simulink model "ForwardKinematic_YuMi"  (R2024a)
(part 21 of 23)

(3148506117433717*sin(q1R))/4503599627370496))/36893488147419103232 + sin(q2R)*((3148506117433717*cos(q1R))/4503599627370496 + (1211728953682539*sin(q1R))/2251799813685248)))/42535295865117307932921825928971026432))/1801439850948198400 - (94754841554645069948206780163139*sin(q5R)*(((7514214926474921*cos(q4R))/36893488147419103232 + (4503599440548691*sin(q4R))/4503599627370496)*((9007199067919185*sin(q3R)*((10914283902180054573281797610715*cos(q1R))/20282409603651670423947251286016 - (28359221366286827792295350160645*sin(q1R))/40564819207303340847894502572032))/9007199254740992 + cos(q3R)*(cos(q2R)*((3148506117433717*cos(q1R))/4503599627370496 + (1211728953682539*sin(q1R))/2251799813685248) - (7514214926474921*sin(q2R)*((1211728953682539*cos(q1R))/2251799813685248 - (3148506117433717*sin(q1R))/4503599627370496))/36893488147419103232) + (7514214926474921*sin(q3R)*((7514214926474921*cos(q2R)*((1211728953682539*cos(q1R))/2251799813685248 - (3148506117433717*sin(q1R))/4503599627370496))/36893488147419103232 + sin(q2R)*((3148506117433717*cos(q1R))/4503599627370496 + (1211728953682539*sin(q1R))/2251799813685248)))/36893488147419103232) + ((9007199067919185*cos(q4R))/9007199254740992 - (234819211581865*sin(q4R))/1152921504606846976)*((213097284493758984364555654519459856780913684045*sin(q1R))/1496577676626844588240573268701473812127674924007424 - (82012275009546312639155898108543355135168378515*cos(q1R))/748288838313422294120286634350736906063837462003712 + (67682029681889335677290557259385*cos(q2R)*((1211728953682539*cos(q1R))/2251799813685248 - (3148506117433717*sin(q1R))/4503599627370496))/332306998946228968225951765070086144 + (9007199067919185*sin(q2R)*((3148506117433717*cos(q1R))/4503599627370496 + (1211728953682539*sin(q1R))/2251799813685248))/9007199254740992) + (7514214926474921*sin(q4R)*((9007199067919185*cos(q3R)*((10914283902180054573281797610715*cos(q1R))/20282409603651670423947251286016 - (28359221366286827792295350160645*sin(q1R))/40564819207303340847894502572032))/9007199254740992 + (7514214926474921*cos(q3R)*((7514214926474921*cos(q2R)*((1211728953682539*cos(q1R))/2251799813685248 - (3148506117433717*sin(q1R))/4503599627370496))/36893488147419103232 + sin(q2R)*((3148506117433717*cos(q1R))/4503599627370496 + (1211728953682539*sin(q1R))/2251799813685248)))/36893488147419103232 - sin(q3R)*(cos(q2R)*((3148506117433717*cos(q1R))/4503599627370496 + (1211728953682539*sin(q1R))/2251799813685248) - (7514214926474921*sin(q2R)*((1211728953682539*cos(q1R))/2251799813685248 - (3148506117433717*sin(q1R))/4503599627370496))/36893488147419103232)))/36893488147419103232))/66461399789245793645190353014017228800 + (584133382113593486367040631332731*cos(q6R)*((965783844824089043900160825489639266458473927649494297144005158508529713680125*cos(q1R))/1042962419883256876169444192465601618458351817556959360325703910069443225478828393565899456512 - (2509452575434582988059840876067412966740105600591515474393999405526015293027875*sin(q1R))/2085924839766513752338888384931203236916703635113918720651407820138886450957656787131798913024 + (9007199067919185*((4503599440548691*cos(q4R))/4503599627370496 - (7514214926474921*sin(q4R))/36893488147419103232)*((9007199067919185*sin(q3R)*((10914283902180054573281797610715*cos(q1R))/20282409603651670423947251286016 - (28359221366286827792295350160645*sin(q1R))/40564819207303340847894502572032))/9007199254740992 + cos(q3R)*(cos(q2R)*((3148506117433717*cos(q1R))/4503599627370496 + (1211728953682539*sin(q1R))/2251799813685248) - (7514214926474921*sin(q2R)*((1211728953682539*cos(q1R))/2251799813685248 - (3148506117433717*sin(q1R))/4503599627370496))/36893488147419103232) + (7514214926474921*sin(q3R)*((7514214926474921*cos(q2R)*((1211728953682539*cos(q1R))/2251799813685248 - (3148506117433717*sin(q1R))/4503599627370496))/36893488147419103232 + sin(q2R)*((3148506117433717*cos(q1R))/4503599627370496 + (1211728953682539*sin(q1R))/2251799813685248)))/36893488147419103232))/9007199254740992 - (9007199067919185*((234819211581865*cos(q4R))/1152921504606846976 + (9007199067919185*sin(q4R))/9007199254740992)*((213097284493758984364555654519459856780913684045*sin(q1R))/1496577676626844588240573268701473812127674924007424 - (82012275009546312639155898108543355135168378515*cos(q1R))/748288838313422294120286634350736906063837462003712 + (67682029681889335677290557259385*cos(q2R)*((1211728953682539*cos(q1R))/2251799813685248 - (3148506117433717*sin(q1R))/4503599627370496))/332306998946228968225951765070086144 + (9007199067919185*sin(q2R)*((3148506117433717*cos(q1R))/4503599627370496 + (1211728953682539*sin(q1R))/2251799813685248))/9007199254740992))/9007199254740992 - (797029601289130257223357069404502671534492977261568326111352375*cos(q2R)*((1211728953682539*cos(q1R))/2251799813685248 - (3148506117433717*sin(q1R))/4503599627370496))/463168356949264781694283940034751631413079938662562256157830336031652518559744 - (106069577339469832923929692356850887620017617375*sin(q2R)*((3148506117433717*cos(q1R))/4503599627370496 + (1211728953682539*sin(q1R))/2251799813685248))/12554203470773361527671578846415332832204710888928069025792 + (67682029681889335677290557259385*cos(q4R)*((9007199067919185*cos(q3R)*((10914283902180054573281797610715*cos(q1R))/20282409603651670423947251286016 - (28359221366286827792295350160645*sin(q1R))/40564819207303340847894502572032))/9007199254740992 + (7514214926474921*cos(q3R)*((7514214926474921*cos(q2R)*((1211728953682539*cos(q1R))/2251799813685248 - (3148506117433717*sin(q1R))/4503599627370496))/36893488147419103232 + sin(q2R)*((3148506117433717*cos(q1R))/4503599627370496 + (1211728953682539*sin(q1R))/2251799813685248)))/36893488147419103232 - sin(q3R)*(cos(q2R)*((3148506117433717*cos(q1R))/4503599627370496 + (1211728953682539*sin(q1R))/2251799813685248) - (7514214926474921*sin(q2R)*((1211728953682539*cos(q1R))/2251799813685248 - (3148506117433717*sin(q1R))/4503599627370496))/36893488147419103232)))/332306998946228968225951765070086144 - (609625514665592237562888769449172969868262801225*cos(q3R)*((10914283902180054573281797610715*cos(q1R))/20282409603651670423947251286016 - (28359221366286827792295350160645*sin(q1R))/40564819207303340847894502572032))/2993155353253689176481146537402947624255349848014848 + (15893040848161638993908057577265778144967053025*sin(q3R)*((10914283902180054573281797610715*cos(q1R))/20282409603651670423947251286016 - (28359221366286827792295350160645*sin(q1R))/40564819207303340847894502572032))/383123885216472214589586756787577295904684780545900544 + (1764482024691522628700660907665*cos(q3R)*(cos(q2R)*((3148506117433717*cos(q1R))/4503599627370496 + (1211728953682539*sin(q1R))/2251799813685248) - (7514214926474921*sin(q2R)*((1211728953682539*cos(q1R))/2251799813685248 - (3148506117433717*sin(q1R))/4503599627370496))/36893488147419103232))/42535295865117307932921825928971026432 - (508577317689771495245073589786522929324694383585*cos(q3R)*((7514214926474921*cos(q2R)*((1211728953682539*cos(q1R))/2251799813685248 - (3148506117433717*sin(q1R))/4503599627370496))/36893488147419103232 + sin(q2R)*((3148506117433717*cos(q1R))/4503599627370496 + (1211728953682539*sin(q1R))/2251799813685248)))/12259964326927110866866776217202473468949912977468817408 + (67682029681889335677290557259385*sin(q3R)*(cos(q2R)*((3148506117433717*cos(q1R))/4503599627370496 + (1211728953682539*sin(q1R))/2251799813685248) - (7514214926474921*sin(q2R)*((1211728953682539*cos(q1R))/2251799813685248 - (3148506117433717*sin(q1R))/4503599627370496))/36893488147419103232))/332306998946228968225951765070086144 + (13258697167433729449897784796786197386719169465*sin(q3R)*((7514214926474921*cos(q2R)*((1211728953682539*cos(q1R))/2251799813685248 - (3148506117433717*sin(q1R))/4503599627370496))/36893488147419103232 + sin(q2R)*((3148506117433717*cos(q1R))/4503599627370496 + (1211728953682539*sin(q1R))/2251799813685248)))/1569275433846670190958947355801916604025588861116008628224))/16225927682921336339157801028812800 + (48638874966763599*sin(q6R)*((965783844824089043900160825489639266458473927649494297144005158508529713680125*cos(q1R))/1042962419883256876169444192465601618458351817556959360325703910069443225478828393565899456512 - (2509452575434582988059840876067412966740105600591515474393999405526015293027875*sin(q1R))/2085924839766513752338888384931203236916703635113918720651407820138886450957656787131798913024 + (9007199067919185*((4503599440548691*cos(q4R))/4503599627370496 - (7514214926474921*sin(q4R))/36893488147419103232)*((9007199067919185*sin(q3R)*((10914283902180054573281797610715*cos(q1R))/20282409603651670423947251286016 - (28359221366286827792295350160645*sin(q1R))/40564819207303340847894502572032))/9007199254740992 + cos(q3R)*(cos(q2R)*((3148506117433717*cos(q1R))/4503599627370496 + (1211728953682539*sin(q1R))/2251799813685248) - (7514214926474921*sin(q2R)*((1211728953682539*cos(q1R))/2251799813685248 - (3148506117433717*sin(q1R))/4503599627370496))/36893488147419103232) + (7514214926474921*sin(q3R)*((7514214926474921*cos(q2R)*((1211728953682539*cos(q1R))/2251799813685248 - (3148506117433717*sin(q1R))/4503599627370496))/36893488147419103232 + sin(q2R)*((3148506117433717*cos(q1R))/4503599627370496 + (1211728953682539*sin(q1R))/2251799813685248)))/36893488147419103232))/9007199254740992 - (9007199067919185*((234819211581865*cos(q4R))/1152921504606846976 + (9007199067919185*sin(q4R))/9007199254740992)*((213097284493758984364555654519459856780913684045*sin(q1R))/1496577676626844588240573268701473812127674924007424 - (82012275009546312639155898108543355135168378515*cos(q1R))/748288838313422294120286634350736906063837462003712 + (67682029681889335677290557259385*cos(q2R)*((1211728953682539*cos(q1R))/2251799813685248 - (3148506117433717*sin(q1R))/4503599627370496))/332306998946228968225951765070086144 + (9007199067919185*sin(q2R)*((3148506117433717*cos(q1R))/4503599627370496 + (1211728953682539*sin(q1R))/2251799813685248))/9007199254740992))/9007199254740992 - (797029601289130257223357069404502671534492977261568326111352375*cos(q2R)*((1211728953682539*cos(q1R))/2251799813685248 - (3148506117433717*sin(q1R))/4503599627370496))/463168356949264781694283940034751631413079938662562256157830336031652518559744 - (106069577339469832923929692356850887620017617375*sin(q2R)*((3148506117433717*cos(q1R))/4503599627370496 + (1211728953682539*sin(q1R))/2251799813685248))/12554203470773361527671578846415332832204710888928069025792 + (67682029681889335677290557259385*cos(q4R)*((9007199067919185*cos(q3R)*((10914283902180054573281797610715*cos(q1R))/20282409603651670423947251286016 - (28359221366286827792295350160645*sin(q1R))/40564819207303340847894502572032))/9007199254740992 + (7514214926474921*cos(q3R)*((7514214926474921*cos(q2R)*((1211728953682539*cos(q1R))/2251799813685248 - (3148506117433717*sin(q1R))/4503599627370496))/36893488147419103232 + sin(q2R)*((3148506117433717*cos(q1R))/4503599627370496 + (1211728953682539*sin(q1R))/2251799813685248)))/36893488147419103232 - sin(q3R)*(cos(q2R)*((3148506117433717*cos(q1R))/4503599627370496 + (1211728953682539*sin(q1R))/2251799813685248) - (7514214926474921*sin(q2R)*((1211728953682539*cos(q1R))/2251799813685248 - (3148506117433717*sin(q1R))/4503599627370496))/36893488147419103232)))/332306998946228968225951765070086144 - (609625514665592237562888769449172969868262801225*cos(q3R)*((10914283902180054573281797610715*cos(q1R))/20282409603651670423947251286016 - (28359221366286827792295350160645*sin(q1R))/40564819207303340847894502572032))/2993155353253689176481146537402947624255349848014848 + (15893040848161638993908057577265778144967053025*sin(q3R)*((10914283902180054573281797610715*cos(q1R))/20282409603651670423947251286016 - (28359221366286827792295350160645*sin(q1R))/40564819207303340847894502572032))/383123885216472214589586756787577295904684780545900544 + (1764482024691522628700660907665*cos(q3R)*(cos(q2R)*((3148506117433717*cos(q1R))/4503599627370496 + (1211728953682539*sin(q1R))/2251799813685248) - (7514214926474921*sin(q2R)*((1211728953682539*cos(q1R))/2251799813685248 - (3148506117433717*sin(q1R))/4503599627370496))/36893488147419103232))/42535295865117307932921825928971026432 - (508577317689771495245073589786522929324694383585*cos(q3R)*((7514214926474921*cos(q2R)*((1211728953682539*cos(q1R))/2251799813685248 - (3148506117433717*sin(q1R))/4503599627370496))/36893488147419103232 + sin(q2R)*((3148506117433717*cos(q1R))/4503599627370496 + (1211728953682539*sin(q1R))/2251799813685248)))/12259964326927110866866776217202473468949912977468817408 + (67682029681889335677290557259385*sin(q3R)*(cos(q2R)*((3148506117433717*cos(q1R))/4503599627370496 + (1211728953682539*sin(q1R))/2251799813685248) - (7514214926474921*sin(q2R)*((1211728953682539*cos(q1R))/2251799813685248 - (3148506117433717*sin(q1R))/4503599627370496))/36893488147419103232))/332306998946228968225951765070086144 + (13258697167433729449897784796786197386719169465*sin(q3R)*((7514214926474921*cos(q2R)*((1211728953682539*cos(q1R))/2251799813685248 - (3148506117433717*sin(q1R))/4503599627370496))/36893488147419103232 + sin(q2R)*((3148506117433717*cos(q1R))/4503599627370496 + (1211728953682539*sin(q1R))/2251799813685248)))/1569275433846670190958947355801916604025588861116008628224))/1801439850948198400 + (610321541873521657855151997354401418608858870661075444886782706002880706727*cos(q4R)*((9007199067919185*cos(q3R)*((10914283902180054573281797610715*cos(q1R))/20282409603651670423947251286016 - (28359221366286827792295350160645*sin(q1R))/40564819207303340847894502572032))/9007199254740992 + (7514214926474921*cos(q3R)*((7514214926474921*cos(q2R)*((1211728953682539*cos(q1R))/2251799813685248 - (3148506117433717*sin(q1R))/4503599627370496))/36893488147419103232 + sin(q2R)*((3148506117433717*cos(q1R))/4503599627370496 + (1211728953682539*sin(q1R))/2251799813685248)))/36893488147419103232 - sin(q3R)*(cos(q2R)*((3148506117433717*cos(q1R))/4503599627370496 + (1211728953682539*sin(q1R))/2251799813685248) - (7514214926474921*sin(q2R)*((1211728953682539*cos(q1R))/2251799813685248 - (3148506117433717*sin(q1R))/4503599627370496))/36893488147419103232)))/11307821214581659709333104004754678501295896940003961331978279688272766566400000 + (608651409044468601*sin(q4R)*((9007199067919185*cos(q3R)*((10914283902180054573281797610715*cos(q1R))/20282409603651670423947251286016 - (28359221366286827792295350160645*sin(q1R))/40564819207303340847894502572032))/9007199254740992 + (7514214926474921*cos(q3R)*((7514214926474921*cos(q2R)*((1211728953682539*cos(q1R))/2251799813685248 - (3148506117433717*sin(q1R))/4503599627370496))/36893488147419103232 + sin(q2R)*((3148506117433717*cos(q1R))/4503599627370496 + (1211728953682539*sin(q1R))/2251799813685248)))/36893488147419103232 - sin(q3R)*(cos(q2R)*((3148506117433717*cos(q1R))/4503599627370496 + (1211728953682539*sin(q1R))/2251799813685248) - (7514214926474921*sin(q2R)*((1211728953682539*cos(q1R))/2251799813685248 - (3148506117433717*sin(q1R))/4503599627370496))/36893488147419103232)))/73786976294838206464000 - (83301539375654672537075965313343183841442266989297270401707771044036658496661398777306991*cos(q3R)*((10914283902180054573281797610715*cos(q1R))/20282409603651670423947251286016 - (28359221366286827792295350160645*sin(q1R))/40564819207303340847894502572032))/4074071952668972172536891376818756322102936787331872501272280898708762599526673412366794752000 + (109198173955282063961996941994332957526645881091499469714283881779231664456243735535448036415347*sin(q3R)*((10914283902180054573281797610715*cos(q1R))/20282409603651670423947251286016 - (28359221366286827792295350160645*sin(q1R))/40564819207303340847894502572032))/2607406049708142190423610481164004046145879543892398400814259775173608063697070983914748641280000 + (60617164743372705924380750591060836759586313939367162716784907429017787816377231*cos(q3R)*(cos(q2R)*((3148506117433717*cos(q1R))/4503599627370496 + (1211728953682539*sin(q1R))/2251799813685248) - (7514214926474921*sin(q2R)*((1211728953682539*cos(q1R))/2251799813685248 - (3148506117433717*sin(q1R))/4503599627370496))/36893488147419103232))/1447401115466452442794637312608598848165874808320507050493219800098914120499200000 - (347469655025336708709976918716104493695816557877713443586884917071777956519687017125887603*cos(q3R)*((7514214926474921*cos(q2R)*((1211728953682539*cos(q1R))/2251799813685248 - (3148506117433717*sin(q1R))/4503599627370496))/36893488147419103232 + sin(q2R)*((3148506117433717*cos(q1R))/4503599627370496 + (1211728953682539*sin(q1R))/2251799813685248)))/83436993590660550093555535397248129476668145404556748826056312805555458038306271485271956520960000 + (46241644459901303158631016767207157814229090534989303509431886332469146043*sin(q3R)*(cos(q2R)*((3148506117433717*cos(q1R))/4503599627370496 + (1211728953682539*sin(q1R))/2251799813685248) - (7514214926474921*sin(q2R)*((1211728953682539*cos(q1R))/2251799813685248 - (3148506117433717*sin(q1R))/4503599627370496))/36893488147419103232))/2261564242916331941866620800950935700259179388000792266395655937654553313280000 + (455490404115240510935077772268745492204390157443214084883134054419271951750419293234291596923751*sin(q3R)*((7514214926474921*cos(q2R)*((1211728953682539*cos(q1R))/2251799813685248 - (3148506117433717*sin(q1R))/4503599627370496))/36893488147419103232 + sin(q2R)*((3148506117433717*cos(q1R))/4503599627370496 + (1211728953682539*sin(q1R))/2251799813685248)))/53399675898022752059875542654238802865067613058916319248676040195555493144516013750574052173414400000, (81222263116692158804177042061221826384594597321566869716687*((234819211581865*cos(q4R))/1152921504606846976 + (9007199067919185*sin(q4R))/9007199254740992)*((43007175577195104036898489188735438973874147925*sin(q2R))/91343852333181432387730302044767688728495783936 + (9007199067919185*cos(q2R)*((1211728953682539*cos(q1R))/2251799813685248 - (3148506117433717*sin(q1R))/4503599627370496))/9007199254740992 + (67682029681889335677290557259385*sin(q2R)*((3148506117433717*cos(q1R))/4503599627370496 + (1211728953682539*sin(q1R))/2251799813685248))/332306998946228968225951765070086144))/306499108173177771671669405430061836723747824436720435200000 - (102624569379093796004717602421110099184671668506065630314089972323079075980539460999909738524689495122204956357382384585416279829311*sin(q2R))/866459279412754643618254432544713657323886586054942679740774868942069158689258007199992001907543618155434753425438616196554424320000 - (610321541873521657855151997354401418608858870661075444886782706002880706727*cos(q4R)*((7514214926474921*cos(q3R)*((4774755754024928798560446539205*sin(q2R))/10141204801825835211973625643008 + cos(q2R)*((1211728953682539*cos(q1R))/2251799813685248 - (3148506117433717*sin(q1R))/4503599627370496) + (7514214926474921*sin(q2R)*((3148506117433717*cos(q1R))/4503599627370496 + (1211728953682539*sin(q1R))/2251799813685248))/36893488147419103232))/36893488147419103232 - sin(q3R)*((4774755754024928798560446539205*cos(q2R))/10141204801825835211973625643008 + (7514214926474921*cos(q2R)*((3148506117433717*cos(q1R))/4503599627370496 + (1211728953682539*sin(q1R))/2251799813685248))/36893488147419103232 - sin(q2R)*((1211728953682539*cos(q1R))/2251799813685248 - (3148506117433717*sin(q1R))/4503599627370496))))/11307821214581659709333104004754678501295896940003961331978279688272766566400000 - (608651409044468601*sin(q4R)*((7514214926474921*cos(q3R)*((4774755754024928798560446539205*sin(q2R))/10141204801825835211973625643008 + cos(q2R)*((1211728953682539*cos(q1R))/2251799813685248 - (3148506117433717*sin(q1R))/4503599627370496) + (7514214926474921*sin(q2R)*((3148506117433717*cos(q1R))/4503599627370496 + (1211728953682539*sin(q1R))/2251799813685248))/36893488147419103232))/36893488147419103232 - sin(q3R)*((4774755754024928798560446539205*cos(q2R))/10141204801825835211973625643008 + (7514214926474921*cos(q2R)*((3148506117433717*cos(q1R))/4503599627370496 + (1211728953682539*sin(q1R))/2251799813685248))/36893488147419103232 - sin(q2R)*((1211728953682539*cos(q1R))/2251799813685248 - (3148506117433717*sin(q1R))/4503599627370496))))/73786976294838206464000 - (81*((9007199067919185*cos(q4R))/9007199254740992 - (234819211581865*sin(q4R))/1152921504606846976)*((43007175577195104036898489188735438973874147925*sin(q2R))/91343852333181432387730302044767688728495783936 + (9007199067919185*cos(q2R)*((1211728953682539*cos(q1R))/2251799813685248 - (3148506117433717*sin(q1R))/4503599627370496))/9007199254740992 + (67682029681889335677290557259385*sin(q2R)*((3148506117433717*cos(q1R))/4503599627370496 + (1211728953682539*sin(q1R))/2251799813685248))/332306998946228968225951765070086144))/2000 - (2864853452414957279136267923523*cos(q2R))/202824096036516704239472512860160 + (170695144106365826517608855445768431563113584343*cos(q5R)*((67399765602155231606998903473897443684277400996768941497011875*sin(q2R))/3450873173395281893717377931138512726225554486085193277581262111899648 + (14115856197532180673579726082375*cos(q2R)*((1211728953682539*cos(q1R))/2251799813685248 - (3148506117433717*sin(q1R))/4503599627370496))/340282366920938463463374607431768211456 - (234819211581865*cos(q3R)*((4774755754024928798560446539205*cos(q2R))/10141204801825835211973625643008 + (7514214926474921*cos(q2R)*((3148506117433717*cos(q1R))/4503599627370496 + (1211728953682539*sin(q1R))/2251799813685248))/36893488147419103232 - sin(q2R)*((1211728953682539*cos(q1R))/2251799813685248 - (3148506117433717*sin(q1R))/4503599627370496)))/1152921504606846976 + (106069577339469832923929692356850887620017617375*sin(q2R)*((3148506117433717*cos(q1R))/4503599627370496 + (1211728953682539*sin(q1R))/2251799813685248))/12554203470773361527671578846415332832204710888928069025792 + (67682029681889335677290557259385*cos(q3R)*((4774755754024928798560446539205*sin(q2R))/10141204801825835211973625643008 + cos(q2R)*((1211728953682539*cos(q1R))/2251799813685248 - (3148506117433717*sin(q1R))/4503599627370496) + (7514214926474921*sin(q2R)*((3148506117433717*cos(q1R))/4503599627370496 + (1211728953682539*sin(q1R))/2251799813685248))/36893488147419103232))/332306998946228968225951765070086144 - (9007199067919185*sin(q3R)*((4774755754024928798560446539205*cos(q2R))/10141204801825835211973625643008 + (7514214926474921*cos(q2R)*((3148506117433717*cos(q1R))/4503599627370496 + (1211728953682539*sin(q1R))/2251799813685248))/36893488147419103232 - sin(q2R)*((1211728953682539*cos(q1R))/2251799813685248 - (3148506117433717*sin(q1R))/4503599627370496)))/9007199254740992 - (1764482024691522628700660907665*sin(q3R)*((4774755754024928798560446539205*sin(q2R))/10141204801825835211973625643008 + cos(q2R)*((1211728953682539*cos(q1R))/2251799813685248 - (3148506117433717*sin(q1R))/4503599627370496) + (7514214926474921*sin(q2R)*((3148506117433717*cos(q1R))/4503599627370496 + (1211728953682539*sin(q1R))/2251799813685248))/36893488147419103232))/42535295865117307932921825928971026432))/119726214130147567059245861496117904970213993920593920 - (48638874966763599*sin(q5R)*((67399765602155231606998903473897443684277400996768941497011875*sin(q2R))/3450873173395281893717377931138512726225554486085193277581262111899648 + (14115856197532180673579726082375*cos(q2R)*((1211728953682539*cos(q1R))/2251799813685248 - (3148506117433717*sin(q1R))/4503599627370496))/340282366920938463463374607431768211456 - (234819211581865*cos(q3R)*((4774755754024928798560446539205*cos(q2R))/10141204801825835211973625643008 + (7514214926474921*cos(q2R)*((3148506117433717*cos(q1R))/4503599627370496 + (1211728953682539*sin(q1R))/2251799813685248))/36893488147419103232 - sin(q2R)*((1211728953682539*cos(q1R))/2251799813685248 - (3148506117433717*sin(q1R))/4503599627370496)))/1152921504606846976 + (106069577339469832923929692356850887620017617375*sin(q2R)*((3148506117433717*cos(q1R))/4503599627370496 + (1211728953682539*sin(q1R))/2251799813685248))/12554203470773361527671578846415332832204710888928069025792 + (67682029681889335677290557259385*cos(q3R)*((4774755754024928798560446539205*sin(q2R))/10141204801825835211973625643008 + cos(q2R)*((1211728953682539*cos(q1R))/2251799813685248 - (3148506117433717*sin(q1R))/4503599627370496) + (7514214926474921*sin(q2R)*((3148506117433717*cos(q1R))/4503599627370496 + (1211728953682539*sin(q1R))/2251799813685248))/36893488147419103232))/332306998946228968225951765070086144 - (9007199067919185*sin(q3R)*((4774755754024928798560446539205*cos(q2R))/10141204801825835211973625643008 + (7514214926474921*cos(q2R)*((3148506117433717*cos(q1R))/4503599627370496 + (1211728953682539*sin(q1R))/2251799813685248))/36893488147419103232 - sin(q2R)*((1211728953682539*cos(q1R))/2251799813685248 - (3148506117433717*sin(q1R))/4503599627370496)))/9007199254740992 - (1764482024691522628700660907665*sin(q3R)*((4774755754024928798560446539205*sin(q2R))/10141204801825835211973625643008 + cos(q2R)*((1211728953682539*cos(q1R))/2251799813685248 - (3148506117433717*sin(q1R))/4503599627370496) + (7514214926474921*sin(q2R)*((3148506117433717*cos(q1R))/4503599627370496 + (1211728953682539*sin(q1R))/2251799813685248))/36893488147419103232))/42535295865117307932921825928971026432))/1801439850948198400 - (107465779053290185796889472867275736954369330186921663479979246519176992895505610212310958309481948671*cos(q2R)*((1211728953682539*cos(q1R))/2251799813685248 - (3148506117433717*sin(q1R))/4503599627370496))/427197407184182016479004341233910422920540904471330553989408321564443945156128110004592417387315200000 - (22542644779424763*cos(q2R)*((3148506117433717*cos(q1R))/4503599627370496 + (1211728953682539*sin(q1R))/2251799813685248))/3689348814741910323200 - (60617164743372705924380750591060836759586313939367162716784907429017787816377231*cos(q3R)*((4774755754024928798560446539205*cos(q2R))/10141204801825835211973625643008 + (7514214926474921*cos(q2R)*((3148506117433717*cos(q1R))/4503599627370496 + (1211728953682539*sin(q1R))/2251799813685248))/36893488147419103232 - sin(q2R)*((1211728953682539*cos(q1R))/2251799813685248 - (3148506117433717*sin(q1R))/4503599627370496)))/1447401115466452442794637312608598848165874808320507050493219800098914120499200000 + (3*sin(q2R)*((1211728953682539*cos(q1R))/2251799813685248 - (3148506117433717*sin(q1R))/4503599627370496))/100 - (807520961047489018778067709720399904923771262077295170375712179706208528987338271217011451790113918662491539890779991*sin(q2R)*((3148506117433717*cos(q1R))/4503599627370496 + (1211728953682539*sin(q1R))/2251799813685248))/15760802478557791684911616040057445522031895708186178667179317361698288708598884244565706501953966256322651196122726400000 + (347469655025336708709976918716104493695816557877713443586884917071777956519687017125887603*cos(q3R)*((4774755754024928798560446539205*sin(q2R))/10141204801825835211973625643008 + cos(q2R)*((1211728953682539*cos(q1R))/2251799813685248 - (3148506117433717*sin(q1R))/4503599627370496) + (7514214926474921*sin(q2R)*((3148506117433717*cos(q1R))/4503599627370496 + (1211728953682539*sin(q1R))/2251799813685248))/36893488147419103232))/83436993590660550093555535397248129476668145404556748826056312805555458038306271485271956520960000 - (46241644459901303158631016767207157814229090534989303509431886332469146043*sin(q3R)*((4774755754024928798560446539205*cos(q2R))/10141204801825835211973625643008 + (7514214926474921*cos(q2R)*((3148506117433717*cos(q1R))/4503599627370496 + (1211728953682539*sin(q1R))/2251799813685248))/36893488147419103232 - sin(q2R)*((1211728953682539*cos(q1R))/2251799813685248 - (3148506117433717*sin(q1R))/4503599627370496)))/2261564242916331941866620800950935700259179388000792266395655937654553313280000 - (81222263116692158804177042061221826384594597321566869716687*((4503599440548691*cos(q4R))/4503599627370496 - (7514214926474921*sin(q4R))/36893488147419103232)*(cos(q3R)*((4774755754024928798560446539205*cos(q2R))/10141204801825835211973625643008 + (7514214926474921*cos(q2R)*((3148506117433717*cos(q1R))/4503599627370496 + (1211728953682539*sin(q1R))/2251799813685248))/36893488147419103232 - sin(q2R)*((1211728953682539*cos(q1R))/2251799813685248 - (3148506117433717*sin(q1R))/4503599627370496)) + (7514214926474921*sin(q3R)*((4774755754024928798560446539205*sin(q2R))/10141204801825835211973625643008 + cos(q2R)*((1211728953682539*cos(q1R))/2251799813685248 - (3148506117433717*sin(q1R))/4503599627370496) + (7514214926474921*sin(q2R)*((3148506117433717*cos(q1R))/4503599627370496 + (1211728953682539*sin(q1R))/2251799813685248))/36893488147419103232))/36893488147419103232))/306499108173177771671669405430061836723747824436720435200000 - (81*((7514214926474921*cos(q4R))/36893488147419103232 + (4503599440548691*sin(q4R))/4503599627370496)*(cos(q3R)*((4774755754024928798560446539205*cos(q2R))/10141204801825835211973625643008 + (7514214926474921*cos(q2R)*((3148506117433717*cos(q1R))/4503599627370496 + (1211728953682539*sin(q1R))/2251799813685248))/36893488147419103232 - sin(q2R)*((1211728953682539*cos(q1R))/2251799813685248 - (3148506117433717*sin(q1R))/4503599627370496)) + (7514214926474921*sin(q3R)*((4774755754024928798560446539205*sin(q2R))/10141204801825835211973625643008 + cos(q2R)*((1211728953682539*cos(q1R))/2251799813685248 - (3148506117433717*sin(q1R))/4503599627370496) + (7514214926474921*sin(q2R)*((3148506117433717*cos(q1R))/4503599627370496 + (1211728953682539*sin(q1R))/2251799813685248))/36893488147419103232))/36893488147419103232))/2000 - (455490404115240510935077772268745492204390157443214084883134054419271951750419293234291596923751*sin(q3R)*((4774755754024928798560446539205*sin(q2R))/10141204801825835211973625643008 + cos(q2R)*((1211728953682539*cos(q1R))/2251799813685248 - (3148506117433717*sin(q1R))/4503599627370496) + (7514214926474921*sin(q2R)*((3148506117433717*cos(q1R))/4503599627370496 + (1211728953682539*sin(q1R))/2251799813685248))/36893488147419103232))/53399675898022752059875542654238802865067613058916319248676040195555493144516013750574052173414400000 + (712008244765680093343103025701132101054572137019*cos(q5R)*((7514214926474921*cos(q4R)*((7514214926474921*cos(q3R)*((4774755754024928798560446539205*sin(q2R))/10141204801825835211973625643008 + cos(q2R)*((1211728953682539*cos(q1R))/2251799813685248 - (3148506117433717*sin(q1R))/4503599627370496) + (7514214926474921*sin(q2R)*((3148506117433717*cos(q1R))/4503599627370496 + (1211728953682539*sin(q1R))/2251799813685248))/36893488147419103232))/36893488147419103232 - sin(q3R)*((4774755754024928798560446539205*cos(q2R))/10141204801825835211973625643008 + (7514214926474921*cos(q2R)*((3148506117433717*cos(q1R))/4503599627370496 + (1211728953682539*sin(q1R))/2251799813685248))/36893488147419103232 - sin(q2R)*((1211728953682539*cos(q1R))/2251799813685248 - (3148506117433717*sin(q1R))/4503599627370496))))/36893488147419103232 - ((234819211581865*cos(q4R))/1152921504606846976 + (9007199067919185*sin(q4R))/9007199254740992)*((43007175577195104036898489188735438973874147925*sin(q2R))/91343852333181432387730302044767688728495783936 + (9007199067919185*cos(q2R)*((1211728953682539*cos(q1R))/2251799813685248 - (3148506117433717*sin(q1R))/4503599627370496))/9007199254740992 + (67682029681889335677290557259385*sin(q2R)*((3148506117433717*cos(q1R))/4503599627370496 + (1211728953682539*sin(q1R))/2251799813685248))/332306998946228968225951765070086144) + ((4503599440548691*cos(q4R))/4503599627370496 - (7514214926474921*sin(q4R))/36893488147419103232)*(cos(q3R)*((4774755754024928798560446539205*cos(q2R))/10141204801825835211973625643008 + (7514214926474921*cos(q2R)*((3148506117433717*cos(q1R))/4503599627370496 + (1211728953682539*sin(q1R))/2251799813685248))/36893488147419103232 - sin(q2R)*((1211728953682539*cos(q1R))/2251799813685248 - (3148506117433717*sin(q1R))/4503599627370496)) + (7514214926474921*sin(q3R)*((4774755754024928798560446539205*sin(q2R))/10141204801825835211973625643008 + cos(q2R)*((1211728953682539*cos(q1R))/2251799813685248 - (3148506117433717*sin(q1R))/4503599627370496) + (7514214926474921*sin(q2R)*((3148506117433717*cos(q1R))/4503599627370496 + (1211728953682539*sin(q1R))/2251799813685248))/36893488147419103232))/36893488147419103232)))/2451992865385422173373355243440494693789982595493763481600 - (2436553109258773196144549622003023*cos(q6R)*((9007199067919185*cos(q5R)*((67399765602155231606998903473897443684277400996768941497011875*sin(q2R))/3450873173395281893717377931138512726225554486085193277581262111899648 + (14115856197532180673579726082375*cos(q2R)*((1211728953682539*cos(q1R))/2251799813685248 - (3148506117433717*sin(q1R))/4503599627370496))/340282366920938463463374607431768211456 - (234819211581865*cos(q3R)*((4774755754024928798560446539205*cos(q2R))/10141204801825835211973625643008 + (7514214926474921*cos(q2R)*((3148506117433717*cos(q1R))/4503599627370496 + (1211728953682539*sin(q1R))/2251799813685248))/36893488147419103232 - sin(q2R)*((1211728953682539*cos(q1R))/2251799813685248 - (3148506117433717*sin(q1R))/4503599627370496)))/1152921504606846976 + (106069577339469832923929692356850887620017617375*sin(q2R)*((3148506117433717*cos(q1R))/4503599627370496 + (1211728953682539*sin(q1R))/2251799813685248))/12554203470773361527671578846415332832204710888928069025792 + (67682029681889335677290557259385*cos(q3R)*((4774755754024928798560446539205*sin(q2R))/10141204801825835211973625643008 + cos(q2R)*((1211728953682539*cos(q1R))/2251799813685248 - (3148506117433717*sin(q1R))/4503599627370496) + (7514214926474921*sin(q2R)*((3148506117433717*cos(q1R))/4503599627370496 + (1211728953682539*sin(q1R))/2251799813685248))/36893488147419103232))/332306998946228968225951765070086144 - (9007199067919185*sin(q3R)*((4774755754024928798560446539205*cos(q2R))/10141204801825835211973625643008 + (7514214926474921*cos(q2R)*((3148506117433717*cos(q1R))/4503599627370496 + (1211728953682539*sin(q1R))/2251799813685248))/36893488147419103232 - sin(q2R)*((1211728953682539*cos(q1R))/2251799813685248 - (3148506117433717*sin(q1R))/4503599627370496)))/9007199254740992 - (1764482024691522628700660907665*sin(q3R)*((4774755754024928798560446539205*sin(q2R))/10141204801825835211973625643008 + cos(q2R)*((1211728953682539*cos(q1R))/2251799813685248 - (3148506117433717*sin(q1R))/4503599627370496) + (7514214926474921*sin(q2R)*((3148506117433717*cos(q1R))/4503599627370496 + (1211728953682539*sin(q1R))/2251799813685248))/36893488147419103232))/42535295865117307932921825928971026432))/9007199254740992 + (7514214926474921*cos(q5R)*((7514214926474921*cos(q4R)*((7514214926474921*cos(q3R)*((4774755754024928798560446539205*sin(q2R))/10141204801825835211973625643008 + cos(q2R)*((1211728953682539*cos(q1R))/2251799813685248 - (3148506117433717*sin(q1R))/4503599627370496) + (7514214926474921*sin(q2R)*((3148506117433717*cos(q1R))/4503599627370496 + (1211728953682539*sin(q1R))/2251799813685248))/36893488147419103232))/36893488147419103232 - sin(q3R)*((4774755754024928798560446539205*cos(q2R))/10141204801825835211973625643008 + (7514214926474921*cos(q2R)*((3148506117433717*cos(q1R))/4503599627370496 + (1211728953682539*sin(q1R))/2251799813685248))/36893488147419103232 - sin(q2R)*((1211728953682539*cos(q1R))/2251799813685248 - (3148506117433717*sin(q1R))/4503599627370496))))/36893488147419103232 - ((234819211581865*cos(q4R))/1152921504606846976 + (9007199067919185*sin(q4R))/9007199254740992)*((43007175577195104036898489188735438973874147925*sin(q2R))/91343852333181432387730302044767688728495783936 + (9007199067919185*cos(q2R)*((1211728953682539*cos(q1R))/2251799813685248 - (3148506117433717*sin(q1R))/4503599627370496))/9007199254740992 + (67682029681889335677290557259385*sin(q2R)*((3148506117433717*cos(q1R))/4503599627370496 + (1211728953682539*sin(q1R))/2251799813685248))/332306998946228968225951765070086144) + ((4503599440548691*cos(q4R))/4503599627370496 - (7514214926474921*sin(q4R))/36893488147419103232)*(cos(q3R)*((4774755754024928798560446539205*cos(q2R))/10141204801825835211973625643008 + (7514214926474921*cos(q2R)*((3148506117433717*cos(q1R))/4503599627370496 + (1211728953682539*sin(q1R))/2251799813685248))/36893488147419103232 - sin(q2R)*((1211728953682539*cos(q1R))/2251799813685248 - (3148506117433717*sin(q1R))/4503599627370496)) + (7514214926474921*sin(q3R)*((4774755754024928798560446539205*sin(q2R))/10141204801825835211973625643008 + cos(q2R)*((1211728953682539*cos(q1R))/2251799813685248 - (3148506117433717*sin(q1R))/4503599627370496) + (7514214926474921*sin(q2R)*((3148506117433717*cos(q1R))/4503599627370496 + (1211728953682539*sin(q1R))/2251799813685248))/36893488147419103232))/36893488147419103232)))/36893488147419103232 + sin(q5R)*((7514214926474921*sin(q4R)*((7514214926474921*cos(q3R)*((4774755754024928798560446539205*sin(q2R))/10141204801825835211973625643008 + cos(q2R)*((1211728953682539*cos(q1R))/2251799813685248 - (3148506117433717*sin(q1R))/4503599627370496) + (7514214926474921*sin(q2R)*((3148506117433717*cos(q1R))/4503599627370496 + (1211728953682539*sin(q1R))/2251799813685248))/36893488147419103232))/36893488147419103232 - sin(q3R)*((4774755754024928798560446539205*cos(q2R))/10141204801825835211973625643008 + (7514214926474921*cos(q2R)*((3148506117433717*cos(q1R))/4503599627370496 + (1211728953682539*sin(q1R))/2251799813685248))/36893488147419103232 - sin(q2R)*((1211728953682539*cos(q1R))/2251799813685248 - (3148506117433717*sin(q1R))/4503599627370496))))/36893488147419103232 + ((9007199067919185*cos(q4R))/9007199254740992 - (234819211581865*sin(q4R))/1152921504606846976)*((43007175577195104036898489188735438973874147925*sin(q2R))/91343852333181432387730302044767688728495783936 + (9007199067919185*cos(q2R)*((1211728953682539*cos(q1R))/2251799813685248 - (3148506117433717*sin(q1R))/4503599627370496))/9007199254740992 + (67682029681889335677290557259385*sin(q2R)*((3148506117433717*cos(q1R))/4503599627370496 + (1211728953682539*sin(q1R))/2251799813685248))/332306998946228968225951765070086144) + ((7514214926474921*cos(q4R))/36893488147419103232 + (4503599440548691*sin(q4R))/4503599627370496)*(cos(q3R)*((4774755754024928798560446539205*cos(q2R))/10141204801825835211973625643008 + (7514214926474921*cos(q2R)*((3148506117433717*cos(q1R))/4503599627370496 + (1211728953682539*sin(q1R))/2251799813685248))/36893488147419103232 - sin(q2R)*((1211728953682539*cos(q1R))/2251799813685248 - (3148506117433717*sin(q1R))/4503599627370496)) + (7514214926474921*sin(q3R)*((4774755754024928798560446539205*sin(q2R))/10141204801825835211973625643008 + cos(q2R)*((1211728953682539*cos(q1R))/2251799813685248 - (3148506117433717*sin(q1R))/4503599627370496) + (7514214926474921*sin(q2R)*((3148506117433717*cos(q1R))/4503599627370496 + (1211728953682539*sin(q1R))/2251799813685248))/36893488147419103232))/36893488147419103232))))/332306998946228968225951765070086144000 + (27*cos(q5R)*((7514214926474921*sin(q4R)*((7514214926474921*cos(q3R)*((4774755754024928798560446539205*sin(q2R))/10141204801825835211973625643008 + cos(q2R)*((1211728953682539*cos(q1R))/2251799813685248 - (3148506117433717*sin(q1R))/4503599627370496) + (7514214926474921*sin(q2R)*((3148506117433717*cos(q1R))/4503599627370496 + (1211728953682539*sin(q1R))/2251799813685248))/36893488147419103232))/36893488147419103232 - sin(q3R)*((4774755754024928798560446539205*cos(q2R))/10141204801825835211973625643008 + (7514214926474921*cos(q2R)*((3148506117433717*cos(q1R))/4503599627370496 + (1211728953682539*sin(q1R))/2251799813685248))/36893488147419103232 - sin(q2R)*((1211728953682539*cos(q1R))/2251799813685248 - (3148506117433717*sin(q1R))/4503599627370496))))/36893488147419103232 + ((9007199067919185*cos(q4R))/9007199254740992 - (234819211581865*sin(q4R))/1152921504606846976)*((43007175577195104036898489188735438973874147925*sin(q2R))/91343852333181432387730302044767688728495783936 + (9007199067919185*cos(q2R)*((1211728953682539*cos(q1R))/2251799813685248 - (3148506117433717*sin(q1R))/4503599627370496))/9007199254740992 + (67682029681889335677290557259385*sin(q2R)*((3148506117433717*cos(q1R))/4503599627370496 + (1211728953682539*sin(q1R))/2251799813685248))/332306998946228968225951765070086144) + ((7514214926474921*cos(q4R))/36893488147419103232 + (4503599440548691*sin(q4R))/4503599627370496)*(cos(q3R)*((4774755754024928798560446539205*cos(q2R))/10141204801825835211973625643008 + (7514214926474921*cos(q2R)*((3148506117433717*cos(q1R))/4503599627370496 + (1211728953682539*sin(q1R))/2251799813685248))/36893488147419103232 - sin(q2R)*((1211728953682539*cos(q1R))/2251799813685248 - (3148506117433717*sin(q1R))/4503599627370496)) + (7514214926474921*sin(q3R)*((4774755754024928798560446539205*sin(q2R))/10141204801825835211973625643008 + cos(q2R)*((1211728953682539*cos(q1R))/2251799813685248 - (3148506117433717*sin(q1R))/4503599627370496) + (7514214926474921*sin(q2R)*((3148506117433717*cos(q1R))/4503599627370496 + (1211728953682539*sin(q1R))/2251799813685248))/36893488147419103232))/36893488147419103232)))/1000 - (202883803014822867*sin(q5R)*((7514214926474921*cos(q4R)*((7514214926474921*cos(q3R)*((4774755754024928798560446539205*sin(q2R))/10141204801825835211973625643008 + cos(q2R)*((1211728953682539*cos(q1R))/2251799813685248 - (3148506117433717*sin(q1R))/4503599627370496) + (7514214926474921*sin(q2R)*((3148506117433717*cos(q1R))/4503599627370496 + (1211728953682539*sin(q1R))/2251799813685248))/36893488147419103232))/36893488147419103232 - sin(q3R)*((4774755754024928798560446539205*cos(q2R))/10141204801825835211973625643008 + (7514214926474921*cos(q2R)*((3148506117433717*cos(q1R))/4503599627370496 + (1211728953682539*sin(q1R))/2251799813685248))/36893488147419103232 - sin(q2R)*((1211728953682539*cos(q1R))/2251799813685248 - (3148506117433717*sin(q1R))/4503599627370496))))/36893488147419103232 - ((234819211581865*cos(q4R))/1152921504606846976 + (9007199067919185*sin(q4R))/9007199254740992)*((43007175577195104036898489188735438973874147925*sin(q2R))/91343852333181432387730302044767688728495783936 + (9007199067919185*cos(q2R)*((1211728953682539*cos(q1R))/2251799813685248 - (3148506117433717*sin(q1R))/4503599627370496))/9007199254740992 + (67682029681889335677290557259385*sin(q2R)*((3148506117433717*cos(q1R))/4503599627370496 + (1211728953682539*sin(q1R))/2251799813685248))/332306998946228968225951765070086144) + ((4503599440548691*cos(q4R))/4503599627370496 - (7514214926474921*sin(q4R))/36893488147419103232)*(cos(q3R)*((4774755754024928798560446539205*cos(q2R))/10141204801825835211973625643008 + (7514214926474921*cos(q2R)*((3148506117433717*cos(q1R))/4503599627370496 + (1211728953682539*sin(q1R))/2251799813685248))/36893488147419103232 - sin(q2R)*((1211728953682539*cos(q1R))/2251799813685248 - (3148506117433717*sin(q1R))/4503599627370496)) + (7514214926474921*sin(q3R)*((4774755754024928798560446539205*sin(q2R))/10141204801825835211973625643008 + cos(q2R)*((1211728953682539*cos(q1R))/2251799813685248 - (3148506117433717*sin(q1R))/4503599627370496) + (7514214926474921*sin(q2R)*((3148506117433717*cos(q1R))/4503599627370496 + (1211728953682539*sin(q1R))/2251799813685248))/36893488147419103232))/36893488147419103232)))/36893488147419103232000 - (202883803014822867*sin(q6R)*((9007199067919185*cos(q5R)*((67399765602155231606998903473897443684277400996768941497011875*sin(q2R))/3450873173395281893717377931138512726225554486085193277581262111899648 + (14115856197532180673579726082375*cos(q2R)*((1211728953682539*cos(q1R))/2251799813685248 - (3148506117433717*sin(q1R))/4503599627370496))/340282366920938463463374607431768211456 - (234819211581865*cos(q3R)*((4774755754024928798560446539205*cos(q2R))/10141204801825835211973625643008 + (7514214926474921*cos(q2R)*((3148506117433717*cos(q1R))/4503599627370496 + (1211728953682539*sin(q1R))/2251799813685248))/36893488147419103232 - sin(q2R)*((1211728953682539*cos(q1R))/2251799813685248 - (3148506117433717*sin(q1R))/4503599627370496)))/1152921504606846976 + (106069577339469832923929692356850887620017617375*sin(q2R)*((3148506117433717*cos(q1R))/4503599627370496 + (1211728953682539*sin(q1R))/2251799813685248))/12554203470773361527671578846415332832204710888928069025792 + (67682029681889335677290557259385*cos(q3R)*((4774755754024928798560446539205*sin(q2R))/10141204801825835211973625643008 + cos(q2R)*((1211728953682539*cos(q1R))/2251799813685248 - (3148506117433717*sin(q1R))/4503599627370496) + (7514214926474921*sin(q2R)*((3148506117433717*cos(q1R))/4503599627370496 + (1211728953682539*sin(q1R))/2251799813685248))/36893488147419103232))/332306998946228968225951765070086144 - (9007199067919185*sin(q3R)*((4774755754024928798560446539205*cos(q2R))/10141204801825835211973625643008 + (7514214926474921*cos(q2R)*((3148506117433717*cos(q1R))/4503599627370496 + (1211728953682539*sin(q1R))/2251799813685248))/36893488147419103232 - sin(q2R)*((1211728953682539*cos(q1R))/2251799813685248 - (3148506117433717*sin(q1R))/4503599627370496)))/9007199254740992 - (1764482024691522628700660907665*sin(q3R)*((4774755754024928798560446539205*sin(q2R))/10141204801825835211973625643008 + cos(q2R)*((1211728953682539*cos(q1R))/2251799813685248 - (3148506117433717*sin(q1R))/4503599627370496) + (7514214926474921*sin(q2R)*((3148506117433717*cos(q1R))/4503599627370496 + (1211728953682539*sin(q1R))/2251799813685248))/36893488147419103232))/42535295865117307932921825928971026432))/9007199254740992 + (7514214926474921*cos(q5R)*((7514214926474921*cos(q4R)*((7514214926474921*cos(q3R)*((4774755754024928798560446539205*sin(q2R))/10141204801825835211973625643008 + cos(q2R)*((1211728953682539*cos(q1R))/2251799813685248 - (3148506117433717*sin(q1R))/4503599627370496) + (7514214926474921*sin(q2R)*((3148506117433717*cos(q1R))/4503599627370496 + (1211728953682539*sin(q1R))/2251799813685248))/36893488147419103232))/36893488147419103232 - sin(q3R)*((4774755754024928798560446539205*cos(q2R))/10141204801825835211973625643008 + (7514214926474921*cos(q2R)*((3148506117433717*cos(q1R))/4503599627370496 + (1211728953682539*sin(q1R))/2251799813685248))/36893488147419103232 - sin(q2R)*((1211728953682539*cos(q1R))/2251799813685248 - (3148506117433717*sin(q1R))/4503599627370496))))/36893488147419103232 - ((234819211581865*cos(q4R))/1152921504606846976 + (9007199067919185*sin(q4R))/9007199254740992)*((43007175577195104036898489188735438973874147925*sin(q2R))/91343852333181432387730302044767688728495783936 + (9007199067919185*cos(q2R)*((1211728953682539*cos(q1R))/2251799813685248 - (3148506117433717*sin(q1R))/4503599627370496))/9007199254740992 + (67682029681889335677290557259385*sin(q2R)*((3148506117433717*cos(q1R))/4503599627370496 + (1211728953682539*sin(q1R))/2251799813685248))/332306998946228968225951765070086144) + ((4503599440548691*cos(q4R))/4503599627370496 - (7514214926474921*sin(q4R))/36893488147419103232)*(cos(q3R)*((4774755754024928798560446539205*cos(q2R))/10141204801825835211973625643008 + (7514214926474921*cos(q2R)*((3148506117433717*cos(q1R))/4503599627370496 + (1211728953682539*sin(q1R))/2251799813685248))/36893488147419103232 - sin(q2R)*((1211728953682539*cos(q1R))/2251799813685248 - (3148506117433717*sin(q1R))/4503599627370496)) + (7514214926474921*sin(q3R)*((4774755754024928798560446539205*sin(q2R))/10141204801825835211973625643008 + cos(q2R)*((1211728953682539*cos(q1R))/2251799813685248 - (3148506117433717*sin(q1R))/4503599627370496) + (7514214926474921*sin(q2R)*((3148506117433717*cos(q1R))/4503599627370496 + (1211728953682539*sin(q1R))/2251799813685248))/36893488147419103232))/36893488147419103232)))/36893488147419103232 + sin(q5R)*((7514214926474921*sin(q4R)*((7514214926474921*cos(q3R)*((4774755754024928798560446539205*sin(q2R))/10141204801825835211973625643008 + cos(q2R)*((1211728953682539*cos(q1R))/2251799813685248 - (3148506117433717*sin(q1R))/4503599627370496) + (7514214926474921*sin(q2R)*((3148506117433717*cos(q1R))/4503599627370496 + (1211728953682539*sin(q1R))/2251799813685248))/36893488147419103232))/36893488147419103232 - sin(q3R)*((4774755754024928798560446539205*cos(q2R))/10141204801825835211973625643008 + (7514214926474921*cos(q2R)*((3148506117433717*cos(q1R))/4503599627370496 + (1211728953682539*sin(q1R))/2251799813685248))/36893488147419103232 - sin(q2R)*((1211728953682539*cos(q1R))/2251799813685248 - (3148506117433717*sin(q1R))/4503599627370496))))/36893488147419103232 + ((9007199067919185*cos(q4R))/9007199254740992 - (234819211581865*sin(q4R))/1152921504606846976)*((43007175577195104036898489188735438973874147925*sin(q2R))/91343852333181432387730302044767688728495783936 + (9007199067919185*cos(q2R)*((1211728953682539*cos(q1R))/2251799813685248 - (3148506117433717*sin(q1R))/4503599627370496))/9007199254740992 + (67682029681889335677290557259385*sin(q2R)*((3148506117433717*cos(q1R))/4503599627370496 + (1211728953682539*sin(q1R))/2251799813685248))/332306998946228968225951765070086144) + ((7514214926474921*cos(q4R))/36893488147419103232 + (4503599440548691*sin(q4R))/4503599627370496)*(cos(q3R)*((4774755754024928798560446539205*cos(q2R))/10141204801825835211973625643008 + (7514214926474921*cos(q2R)*((3148506117433717*cos(q1R))/4503599627370496 + (1211728953682539*sin(q1R))/2251799813685248))/36893488147419103232 - sin(q2R)*((1211728953682539*cos(q1R))/2251799813685248 - (3148506117433717*sin(q1R))/4503599627370496)) + (7514214926474921*sin(q3R)*((4774755754024928798560446539205*sin(q2R))/10141204801825835211973625643008 + cos(q2R)*((1211728953682539*cos(q1R))/2251799813685248 - (3148506117433717*sin(q1R))/4503599627370496) + (7514214926474921*sin(q2R)*((3148506117433717*cos(q1R))/4503599627370496 + (1211728953682539*sin(q1R))/2251799813685248))/36893488147419103232))/36893488147419103232))))/36893488147419103232000 + (27*cos(q6R)*((9007199067919185*sin(q5R)*((67399765602155231606998903473897443684277400996768941497011875*sin(q2R))/3450873173395281893717377931138512726225554486085193277581262111899648 + (14115856197532180673579726082375*cos(q2R)*((1211728953682539*cos(q1R))/2251799813685248 - (3148506117433717*sin(q1R))/4503599627370496))/340282366920938463463374607431768211456 - (234819211581865*cos(q3R)*((4774755754024928798560446539205*cos(q2R))/10141204801825835211973625643008 + (7514214926474921*cos(q2R)*((3148506117433717*cos(q1R))/4503599627370496 + (1211728953682539*sin(q1R))/2251799813685248))/36893488147419103232 - sin(q2R)*((1211728953682539*cos(q1R))/2251799813685248 - (3148506117433717*sin(q1R))/4503599627370496)))/1152921504606846976 + (106069577339469832923929692356850887620017617375*sin(q2R)*((3148506117433717*cos(q1R))/4503599627370496 + (1211728953682539*sin(q1R))/2251799813685248))/12554203470773361527671578846415332832204710888928069025792 + (67682029681889335677290557259385*cos(q3R)*((4774755754024928798560446539205*sin(q2R))/10141204801825835211973625643008 + cos(q2R)*((1211728953682539*cos(q1R))/2251799813685248 - (3148506117433717*sin(q1R))/4503599627370496) + (7514214926474921*sin(q2R)*((3148506117433717*cos(q1R))/4503599627370496 + (1211728953682539*sin(q1R))/2251799813685248))/36893488147419103232))/332306998946228968225951765070086144 - (9007199067919185*sin(q3R)*((4774755754024928798560446539205*cos(q2R))/10141204801825835211973625643008 + (7514214926474921*cos(q2R)*((3148506117433717*cos(q1R))/4503599627370496 + (1211728953682539*sin(q1R))/2251799813685248))/36893488147419103232 - sin(q2R)*((1211728953682539*cos(q1R))/2251799813685248 - (3148506117433717*sin(q1R))/4503599627370496)))/9007199254740992 - (1764482024691522628700660907665*sin(q3R)*((4774755754024928798560446539205*sin(q2R))/10141204801825835211973625643008 + cos(q2R)*((1211728953682539*cos(q1R))/2251799813685248 - (3148506117433717*sin(q1R))/4503599627370496) + (7514214926474921*sin(q2R)*((3148506117433717*cos(q1R))/4503599627370496 + (1211728953682539*sin(q1R))/2251799813685248))/36893488147419103232))/42535295865117307932921825928971026432))/9007199254740992 - cos(q5R)*((7514214926474921*sin(q4R)*((7514214926474921*cos(q3R)*((4774755754024928798560446539205*sin(q2R))/10141204801825835211973625643008 + cos(q2R)*((1211728953682539*cos(q1R))/2251799813685248 - (3148506117433717*sin(q1R))/4503599627370496) + (7514214926474921*sin(q2R)*((3148506117433717*cos(q1R))/4503599627370496 + (1211728953682539*sin(q1R))/2251799813685248))/36893488147419103232))/36893488147419103232 - sin(q3R)*((4774755754024928798560446539205*cos(q2R))/10141204801825835211973625643008 + (7514214926474921*cos(q2R)*((3148506117433717*cos(q1R))/4503599627370496 + (1211728953682539*sin(q1R))/2251799813685248))/36893488147419103232 - sin(q2R)*((1211728953682539*cos(q1R))/2251799813685248 - (3148506117433717*sin(q1R))/4503599627370496))))/36893488147419103232 + ((9007199067919185*cos(q4R))/9007199254740992 - (234819211581865*sin(q4R))/1152921504606846976)*((43007175577195104036898489188735438973874147925*sin(q2R))/91343852333181432387730302044767688728495783936 + (9007199067919185*cos(q2R)*((1211728953682539*cos(q1R))/2251799813685248 - (3148506117433717*sin(q1R))/4503599627370496))/9007199254740992 + (67682029681889335677290557259385*sin(q2R)*((3148506117433717*cos(q1R))/4503599627370496 + (1211728953682539*sin(q1R))/2251799813685248))/332306998946228968225951765070086144) + ((7514214926474921*cos(q4R))/36893488147419103232 + (4503599440548691*sin(q4R))/4503599627370496)*(cos(q3R)*((4774755754024928798560446539205*cos(q2R))/10141204801825835211973625643008 + (7514214926474921*cos(q2R)*((3148506117433717*cos(q1R))/4503599627370496 + (1211728953682539*sin(q1R))/2251799813685248))/36893488147419103232 - sin(q2R)*((1211728953682539*cos(q1R))/2251799813685248 - (3148506117433717*sin(q1R))/4503599627370496)) + (7514214926474921*sin(q3R)*((4774755754024928798560446539205*sin(q2R))/10141204801825835211973625643008 + cos(q2R)*((1211728953682539*cos(q1R))/2251799813685248 - (3148506117433717*sin(q1R))/4503599627370496) + (7514214926474921*sin(q2R)*((3148506117433717*cos(q1R))/4503599627370496 + (1211728953682539*sin(q1R))/2251799813685248))/36893488147419103232))/36893488147419103232)) + (7514214926474921*sin(q5R)*((7514214926474921*cos(q4R)*((7514214926474921*cos(q3R)*((4774755754024928798560446539205*sin(q2R))/10141204801825835211973625643008 + cos(q2R)*((1211728953682539*cos(q1R))/2251799813685248 - (3148506117433717*sin(q1R))/4503599627370496) + (7514214926474921*sin(q2R)*((3148506117433717*cos(q1R))/4503599627370496 + (1211728953682539*sin(q1R))/2251799813685248))/36893488147419103232))/36893488147419103232 - sin(q3R)*((4774755754024928798560446539205*cos(q2R))/10141204801825835211973625643008 + (7514214926474921*cos(q2R)*((3148506117433717*cos(q1R))/4503599627370496 + (1211728953682539*sin(q1R))/2251799813685248))/36893488147419103232 - sin(q2R)*((1211728953682539*cos(q1R))/2251799813685248 - (3148506117433717*sin(q1R))/4503599627370496))))/36893488147419103232 - ((234819211581865*cos(q4R))/1152921504606846976 + (9007199067919185*sin(q4R))/9007199254740992)*((43007175577195104036898489188735438973874147925*sin(q2R))/91343852333181432387730302044767688728495783936 + (9007199067919185*cos(q2R)*((1211728953682539*cos(q1R))/2251799813685248 - (3148506117433717*sin(q1R))/4503599627370496))/9007199254740992 + (67682029681889335677290557259385*sin(q2R)*((3148506117433717*cos(q1R))/4503599627370496 + (1211728953682539*sin(q1R))/2251799813685248))/332306998946228968225951765070086144) + ((4503599440548691*cos(q4R))/4503599627370496 - (7514214926474921*sin(q4R))/36893488147419103232)*(cos(q3R)*((4774755754024928798560446539205*cos(q2R))/10141204801825835211973625643008 + (7514214926474921*cos(q2R)*((3148506117433717*cos(q1R))/4503599627370496 + (1211728953682539*sin(q1R))/2251799813685248))/36893488147419103232 - sin(q2R)*((1211728953682539*cos(q1R))/2251799813685248 - (3148506117433717*sin(q1R))/4503599627370496)) + (7514214926474921*sin(q3R)*((4774755754024928798560446539205*sin(q2R))/10141204801825835211973625643008 + cos(q2R)*((1211728953682539*cos(q1R))/2251799813685248 - (3148506117433717*sin(q1R))/4503599627370496) + (7514214926474921*sin(q2R)*((3148506117433717*cos(q1R))/4503599627370496 + (1211728953682539*sin(q1R))/2251799813685248))/36893488147419103232))/36893488147419103232)))/36893488147419103232))/1000 + (584133382113593486367040631332731*cos(q6R)*((506456324728625783189839291299220948962368525946389165528853917988948626686875*sin(q2R))/127314748520905380391777855525586135065716774604121015664758778084648831235208544136462336 - (67682029681889335677290557259385*cos(q4R)*((7514214926474921*cos(q3R)*((4774755754024928798560446539205*sin(q2R))/10141204801825835211973625643008 + cos(q2R)*((1211728953682539*cos(q1R))/2251799813685248 - (3148506117433717*sin(q1R))/4503599627370496) + (7514214926474921*sin(q2R)*((3148506117433717*cos(q1R))/4503599627370496 + (1211728953682539*sin(q1R))/2251799813685248))/36893488147419103232))/36893488147419103232 - sin(q3R)*((4774755754024928798560446539205*cos(q2R))/10141204801825835211973625643008 + (7514214926474921*cos(q2R)*((3148506117433717*cos(q1R))/4503599627370496 + (1211728953682539*sin(q1R))/2251799813685248))/36893488147419103232 - sin(q2R)*((1211728953682539*cos(q1R))/2251799813685248 - (3148506117433717*sin(q1R))/4503599627370496))))/332306998946228968225951765070086144 + (9007199067919185*((234819211581865*cos(q4R))/1152921504606846976 + (9007199067919185*sin(q4R))/9007199254740992)*((43007175577195104036898489188735438973874147925*sin(q2R))/91343852333181432387730302044767688728495783936 + (9007199067919185*cos(q2R)*((1211728953682539*cos(q1R))/2251799813685248 - (3148506117433717*sin(q1R))/4503599627370496))/9007199254740992 + (67682029681889335677290557259385*sin(q2R)*((3148506117433717*cos(q1R))/4503599627370496 + (1211728953682539*sin(q1R))/2251799813685248))/332306998946228968225951765070086144))/9007199254740992 + (106069577339469832923929692356850887620017617375*cos(q2R)*((1211728953682539*cos(q1R))/2251799813685248 - (3148506117433717*sin(q1R))/4503599627370496))/12554203470773361527671578846415332832204710888928069025792 - (1764482024691522628700660907665*cos(q3R)*((4774755754024928798560446539205*cos(q2R))/10141204801825835211973625643008 + (7514214926474921*cos(q2R)*((3148506117433717*cos(q1R))/4503599627370496 + (1211728953682539*sin(q1R))/2251799813685248))/36893488147419103232 - sin(q2R)*((1211728953682539*cos(q1R))/2251799813685248 - (3148506117433717*sin(q1R))/4503599627370496)))/42535295865117307932921825928971026432 + (797029601289130257223357069404502671534492977261568326111352375*sin(q2R)*((3148506117433717*cos(q1R))/4503599627370496 + (1211728953682539*sin(q1R))/2251799813685248))/463168356949264781694283940034751631413079938662562256157830336031652518559744 + (508577317689771495245073589786522929324694383585*cos(q3R)*((4774755754024928798560446539205*sin(q2R))/10141204801825835211973625643008 + cos(q2R)*((1211728953682539*cos(q1R))/2251799813685248 - (3148506117433717*sin(q1R))/4503599627370496) + (7514214926474921*sin(q2R)*((3148506117433717*cos(q1R))/4503599627370496 + (1211728953682539*sin(q1R))/2251799813685248))/36893488147419103232))/12259964326927110866866776217202473468949912977468817408 - (67682029681889335677290557259385*sin(q3R)*((4774755754024928798560446539205*cos(q2R))/10141204801825835211973625643008 + (7514214926474921*cos(q2R)*((3148506117433717*cos(q1R))/4503599627370496 + (1211728953682539*sin(q1R))/2251799813685248))/36893488147419103232 - sin(q2R)*((1211728953682539*cos(q1R))/2251799813685248 - (3148506117433717*sin(q1R))/4503599627370496)))/332306998946228968225951765070086144 - (9007199067919185*((4503599440548691*cos(q4R))/4503599627370496 - (7514214926474921*sin(q4R))/36893488147419103232)*(cos(q3R)*((4774755754024928798560446539205*cos(q2R))/10141204801825835211973625643008 + (7514214926474921*cos(q2R)*((3148506117433717*cos(q1R))/4503599627370496 + (1211728953682539*sin(q1R))/2251799813685248))/36893488147419103232 - sin(q2R)*((1211728953682539*cos(q1R))/2251799813685248 - (3148506117433717*sin(q1R))/4503599627370496)) + (7514214926474921*sin(q3R)*((4774755754024928798560446539205*sin(q2R))/10141204801825835211973625643008 + cos(q2R)*((1211728953682539*cos(q1R))/2251799813685248 - (3148506117433717*sin(q1R))/4503599627370496) + (7514214926474921*sin(q2R)*((3148506117433717*cos(q1R))/4503599627370496 + (1211728953682539*sin(q1R))/2251799813685248))/36893488147419103232))/36893488147419103232))/9007199254740992 - (13258697167433729449897784796786197386719169465*sin(q3R)*((4774755754024928798560446539205*sin(q2R))/10141204801825835211973625643008 + cos(q2R)*((1211728953682539*cos(q1R))/2251799813685248 - (3148506117433717*sin(q1R))/4503599627370496) + (7514214926474921*sin(q2R)*((3148506117433717*cos(q1R))/4503599627370496 + (1211728953682539*sin(q1R))/2251799813685248))/36893488147419103232))/1569275433846670190958947355801916604025588861116008628224))/16225927682921336339157801028812800 + (94754841554645069948206780163139*sin(q5R)*((7514214926474921*sin(q4R)*((7514214926474921*cos(q3R)*((4774755754024928798560446539205*sin(q2R))/10141204801825835211973625643008 + cos(q2R)*((1211728953682539*cos(q1R))/2251799813685248 - (3148506117433717*sin(q1R))/4503599627370496) + (7514214926474921*sin(q2R)*((3148506117433717*cos(q1R))/4503599627370496 + (1211728953682539*sin(q1R))/2251799813685248))/36893488147419103232))/36893488147419103232 - sin(q3R)*((4774755754024928798560446539205*cos(q2R))/10141204801825835211973625643008 + (7514214926474921*cos(q2R)*((3148506117433717*cos(q1R))/4503599627370496 + (1211728953682539*sin(q1R))/2251799813685248))/36893488147419103232 - sin(q2R)*((1211728953682539*cos(q1R))/2251799813685248 - (3148506117433717*sin(q1R))/4503599627370496))))/36893488147419103232 + ((9007199067919185*cos(q4R))/9007199254740992 - (234819211581865*sin(q4R))/1152921504606846976)*((43007175577195104036898489188735438973874147925*sin(q2R))/91343852333181432387730302044767688728495783936 + (9007199067919185*cos(q2R)*((1211728953682539*cos(q1R))/2251799813685248 - (3148506117433717*sin(q1R))/4503599627370496))/9007199254740992 + (67682029681889335677290557259385*sin(q2R)*((3148506117433717*cos(q1R))/4503599627370496 + (1211728953682539*sin(q1R))/2251799813685248))/332306998946228968225951765070086144) + ((7514214926474921*cos(q4R))/36893488147419103232 + (4503599440548691*sin(q4R))/4503599627370496)*(cos(q3R)*((4774755754024928798560446539205*cos(q2R))/10141204801825835211973625643008 + (7514214926474921*cos(q2R)*((3148506117433717*cos(q1R))/4503599627370496 + (1211728953682539*sin(q1R))/2251799813685248))/36893488147419103232 - sin(q2R)*((1211728953682539*cos(q1R))/2251799813685248 - (3148506117433717*sin(q1R))/4503599627370496)) + (7514214926474921*sin(q3R)*((4774755754024928798560446539205*sin(q2R))/10141204801825835211973625643008 + cos(q2R)*((1211728953682539*cos(q1R))/2251799813685248 - (3148506117433717*sin(q1R))/4503599627370496) + (7514214926474921*sin(q2R)*((3148506117433717*cos(q1R))/4503599627370496 + (1211728953682539*sin(q1R))/2251799813685248))/36893488147419103232))/36893488147419103232)))/66461399789245793645190353014017228800 - (324259171862923063*sin(q6R)*((9007199067919185*sin(q5R)*((67399765602155231606998903473897443684277400996768941497011875*sin(q2R))/3450873173395281893717377931138512726225554486085193277581262111899648 + (14115856197532180673579726082375*cos(q2R)*((1211728953682539*cos(q1R))/2251799813685248 - (3148506117433717*sin(q1R))/4503599627370496))/340282366920938463463374607431768211456 - (234819211581865*cos(q3R)*((4774755754024928798560446539205*cos(q2R))/10141204801825835211973625643008 + (7514214926474921*cos(q2R)*((3148506117433717*cos(q1R))/4503599627370496 + (1211728953682539*sin(q1R))/2251799813685248))/36893488147419103232 - sin(q2R)*((1211728953682539*cos(q1R))/2251799813685248 - (3148506117433717*sin(q1R))/4503599627370496)))/1152921504606846976 + (106069577339469832923929692356850887620017617375*sin(q2R)*((3148506117433717*cos(q1R))/4503599627370496 + (1211728953682539*sin(q1R))/2251799813685248))/12554203470773361527671578846415332832204710888928069025792 + (67682029681889335677290557259385*cos(q3R)*((4774755754024928798560446539205*sin(q2R))/10141204801825835211973625643008 + cos(q2R)*((1211728953682539*cos(q1R))/2251799813685248 - (3148506117433717*sin(q1R))/4503599627370496) + (7514214926474921*sin(q2R)*((3148506117433717*cos(q1R))/4503599627370496 + (1211728953682539*sin(q1R))/2251799813685248))/36893488147419103232))/332306998946228968225951765070086144 - (9007199067919185*sin(q3R)*((4774755754024928798560446539205*cos(q2R))/10141204801825835211973625643008 + (7514214926474921*cos(q2R)*((3148506117433717*cos(q1R))/4503599627370496 + (1211728953682539*sin(q1R))/2251799813685248))/36893488147419103232 - sin(q2R)*((1211728953682539*cos(q1R))/2251799813685248 - (3148506117433717*sin(q1R))/4503599627370496)))/9007199254740992 - (1764482024691522628700660907665*sin(q3R)*((4774755754024928798560446539205*sin(q2R))/10141204801825835211973625643008 + cos(q2R)*((1211728953682539*cos(q1R))/2251799813685248 - (3148506117433717*sin(q1R))/4503599627370496) + (7514214926474921*sin(q2R)*((3148506117433717*cos(q1R))/4503599627370496 + (1211728953682539*sin(q1R))/2251799813685248))/36893488147419103232))/42535295865117307932921825928971026432))/9007199254740992 - cos(q5R)*((7514214926474921*sin(q4R)*((7514214926474921*cos(q3R)*((4774755754024928798560446539205*sin(q2R))/10141204801825835211973625643008 + cos(q2R)*((1211728953682539*cos(q1R))/2251799813685248 - (3148506117433717*sin(q1R))/4503599627370496) + (7514214926474921*sin(q2R)*((3148506117433717*cos(q1R))/4503599627370496 + (1211728953682539*sin(q1R))/2251799813685248))/36893488147419103232))/36893488147419103232 - sin(q3R)*((4774755754024928798560446539205*cos(q2R))/10141204801825835211973625643008 + (7514214926474921*cos(q2R)*((3148506117433717*cos(q1R))/4503599627370496 + (1211728953682539*sin(q1R))/2251799813685248))/36893488147419103232 - sin(q2R)*((1211728953682539*cos(q1R))/2251799813685248 - (3148506117433717*sin(q1R))/4503599627370496))))/36893488147419103232 + ((9007199067919185*cos(q4R))/9007199254740992 - (234819211581865*sin(q4R))/1152921504606846976)*((43007175577195104036898489188735438973874147925*sin(q2R))/91343852333181432387730302044767688728495783936 + (9007199067919185*cos(q2R)*((1211728953682539*cos(q1R))/2251799813685248 - (3148506117433717*sin(q1R))/4503599627370496))/9007199254740992 + (67682029681889335677290557259385*sin(q2R)*((3148506117433717*cos(q1R))/4503599627370496 + (1211728953682539*sin(q1R))/2251799813685248))/332306998946228968225951765070086144) + ((7514214926474921*cos(q4R))/36893488147419103232 + (4503599440548691*sin(q4R))/4503599627370496)*(cos(q3R)*((4774755754024928798560446539205*cos(q2R))/10141204801825835211973625643008 + (7514214926474921*cos(q2R)*((3148506117433717*cos(q1R))/4503599627370496 + (1211728953682539*sin(q1R))/2251799813685248))/36893488147419103232 - sin(q2R)*((1211728953682539*cos(q1R))/2251799813685248 - (3148506117433717*sin(q1R))/4503599627370496)) + (7514214926474921*sin(q3R)*((4774755754024928798560446539205*sin(q2R))/10141204801825835211973625643008 + cos(q2R)*((1211728953682539*cos(q1R))/2251799813685248 - (3148506117433717*sin(q1R))/4503599627370496) + (7514214926474921*sin(q2R)*((3148506117433717*cos(q1R))/4503599627370496 + (1211728953682539*sin(q1R))/2251799813685248))/36893488147419103232))/36893488147419103232)) + (7514214926474921*sin(q5R)*((7514214926474921*cos(q4R)*((7514214926474921*cos(q3R)*((4774755754024928798560446539205*sin(q2R))/10141204801825835211973625643008 + cos(q2R)*((1211728953682539*cos(q1R))/2251799813685248 - (3148506117433717*sin(q1R))/4503599627370496) + (7514214926474921*sin(q2R)*((3148506117433717*cos(q1R))/4503599627370496 + (1211728953682539*sin(q1R))/2251799813685248))/36893488147419103232))/36893488147419103232 - sin(q3R)*((4774755754024928798560446539205*cos(q2R))/10141204801825835211973625643008 + (7514214926474921*cos(q2R)*((3148506117433717*cos(q1R))/4503599627370496 + (1211728953682539*sin(q1R))/2251799813685248))/36893488147419103232 - sin(q2R)*((1211728953682539*cos(q1R))/2251799813685248 - (3148506117433717*sin(q1R))/4503599627370496))))/36893488147419103232 - ((234819211581865*cos(q4R))/1152921504606846976 + (9007199067919185*sin(q4R))/9007199254740992)*((43007175577195104036898489188735438973874147925*sin(q2R))/91343852333181432387730302044767688728495783936 + (9007199067919185*cos(q2R)*((1211728953682539*cos(q1R))/2251799813685248 - (3148506117433717*sin(q1R))/4503599627370496))/9007199254740992 + (67682029681889335677290557259385*sin(q2R)*((3148506117433717*cos(q1R))/4503599627370496 + (1211728953682539*sin(q1R))/2251799813685248))/332306998946228968225951765070086144) + ((4503599440548691*cos(q4R))/4503599627370496 - (7514214926474921*sin(q4R))/36893488147419103232)*(cos(q3R)*((4774755754024928798560446539205*cos(q2R))/10141204801825835211973625643008 + (7514214926474921*cos(q2R)*((3148506117433717*cos(q1R))/4503599627370496 + (1211728953682539*sin(q1R))/2251799813685248))/36893488147419103232 - sin(q2R)*((1211728953682539*cos(q1R))/2251799813685248 - (3148506117433717*sin(q1R))/4503599627370496)) + (7514214926474921*sin(q3R)*((4774755754024928798560446539205*sin(q2R))/10141204801825835211973625643008 + cos(q2R)*((1211728953682539*cos(q1R))/2251799813685248 - (3148506117433717*sin(q1R))/4503599627370496) + (7514214926474921*sin(q2R)*((3148506117433717*cos(q1R))/4503599627370496 + (1211728953682539*sin(q1R))/2251799813685248))/36893488147419103232))/36893488147419103232)))/36893488147419103232))/9007199254740992000 + (48638874966763599*sin(q6R)*((506456324728625783189839291299220948962368525946389165528853917988948626686875*sin(q2R))/127314748520905380391777855525586135065716774604121015664758778084648831235208544136462336 - (67682029681889335677290557259385*cos(q4R)*((7514214926474921*cos(q3R)*((4774755754024928798560446539205*sin(q2R))/10141204801825835211973625643008 + cos(q2R)*((1211728953682539*cos(q1R))/2251799813685248 - (3148506117433717*sin(q1R))/4503599627370496) + (7514214926474921*sin(q2R)*((3148506117433717*cos(q1R))/4503599627370496 + (1211728953682539*sin(q1R))/2251799813685248))/36893488147419103232))/36893488147419103232 - sin(q3R)*((4774755754024928798560446539205*cos(q2R))/10141204801825835211973625643008 + (7514214926474921*cos(q2R)*((3148506117433717*cos(q1R))/4503599627370496 + (1211728953682539*sin(q1R))/2251799813685248))/36893488147419103232 - sin(q2R)*((1211728953682539*cos(q1R))/2251799813685248 - (3148506117433717*sin(q1R))/4503599627370496))))/332306998946228968225951765070086144 + (9007199067919185*((234819211581865*cos(q4R))/1152921504606846976 + (9007199067919185*sin(q4R))/9007199254740992)*((43007175577195104036898489188735438973874147925*sin(q2R))/91343852333181432387730302044767688728495783936 + (9007199067919185*cos(q2R)*((1211728953682539*cos(q1R))/2251799813685248 - (3148506117433717*sin(q1R))/4503599627370496))/9007199254740992 + (67682029681889335677290557259385*sin(q2R)*((3148506117433717*cos(q1R))/4503599627370496 + (1211728953682539*sin(q1R))/2251799813685248))/332306998946228968225951765070086144))/9007199254740992 + (106069577339469832923929692356850887620017617375*cos(q2R)*((1211728953682539*cos(q1R))/2251799813685248 - (3148506117433717*sin(q1R))/4503599627370496))/12554203470773361527671578846415332832204710888928069025792 - (1764482024691522628700660907665*cos(q3R)*((4774755754024928798560446539205*cos(q2R))/10141204801825835211973625643008 + (7514214926474921*cos(q2R)*((3148506117433717*cos(q1R))/4503599627370496 + (1211728953682539*sin(q1R))/2251799813685248))/36893488147419103232 - sin(q2R)*((1211728953682539*cos(q1R))/2251799813685248 - (3148506117433717*sin(q1R))/4503599627370496)))/42535295865117307932921825928971026432 + (797029601289130257223357069404502671534492977261568326111352375*sin(q2R)*((3148506117433717*cos(q1R))/4503599627370496 + (1211728953682539*sin(q1R))/2251799813685248))/463168356949264781694283940034751631413079938662562256157830336031652518559744 + (508577317689771495245073589786522929324694383585*cos(q3R)*((4774755754024928798560446539205*sin(q2R))/10141204801825835211973625643008 + cos(q2R)*((1211728953682539*cos(q1R))/2251799813685248 - (3148506117433717*sin(q1R))/4503599627370496) + (7514214926474921*sin(q2R)*((3148506117433717*cos(q1R))/4503599627370496 + (1211728953682539*sin(q1R))/2251799813685248))/36893488147419103232))/12259964326927110866866776217202473468949912977468817408 - (67682029681889335677290557259385*sin(q3R)*((4774755754024928798560446539205*cos(q2R))/10141204801825835211973625643008 + (7514214926474921*cos(q2R)*((3148506117433717*cos(q1R))/4503599627370496 + (1211728953682539*sin(q1R))/2251799813685248))/36893488147419103232 - sin(q2R)*((1211728953682539*cos(q1R))/2251799813685248 - (3148506117433717*sin(q1R))/4503599627370496)))/332306998946228968225951765070086144 - (9007199067919185*((4503599440548691*cos(q4R))/4503599627370496 - (7514214926474921*sin(q4R))/36893488147419103232)*(cos(q3R)*((4774755754024928798560446539205*cos(q2R))/10141204801825835211973625643008 + (7514214926474921*cos(q2R)*((3148506117433717*cos(q1R))/4503599627370496 + (1211728953682539*sin(q1R))/2251799813685248))/36893488147419103232 - sin(q2R)*((1211728953682539*cos(q1R))/2251799813685248 - (3148506117433717*sin(q1R))/4503599627370496)) + (7514214926474921*sin(q3R)*((4774755754024928798560446539205*sin(q2R))/10141204801825835211973625643008 + cos(q2R)*((1211728953682539*cos(q1R))/2251799813685248 - (3148506117433717*sin(q1R))/4503599627370496) + (7514214926474921*sin(q2R)*((3148506117433717*cos(q1R))/4503599627370496 + (1211728953682539*sin(q1R))/2251799813685248))/36893488147419103232))/36893488147419103232))/9007199254740992 - (13258697167433729449897784796786197386719169465*sin(q3R)*((4774755754024928798560446539205*sin(q2R))/10141204801825835211973625643008 + cos(q2R)*((1211728953682539*cos(q1R))/2251799813685248 - (3148506117433717*sin(q1R))/4503599627370496) + (7514214926474921*sin(q2R)*((3148506117433717*cos(q1R))/4503599627370496 + (1211728953682539*sin(q1R))/2251799813685248))/36893488147419103232))/1569275433846670190958947355801916604025588861116008628224))/1801439850948198400, (81222263116692158804177042061221826384594597321566869716687*((4503599440548691*cos(q4R))/4503599627370496 - (7514214926474921*sin(q4R))/36893488147419103232)*((7514214926474921*cos(q3R)*((4774755754024928798560446539205*cos(q2R))/10141204801825835211973625643008 + (7514214926474921*cos(q2R)*((3148506117433717*cos(q1R))/4503599627370496 + (1211728953682539*sin(q1R))/2251799813685248))/36893488147419103232 - sin(q2R)*((1211728953682539*cos(q1R))/2251799813685248 - (3148506117433717*sin(q1R))/4503599627370496)))/36893488147419103232 + sin(q3R)*((4774755754024928798560446539205*sin(q2R))/10141204801825835211973625643008 + cos(q2R)*((1211728953682539*cos(q1R))/2251799813685248 - (3148506117433717*sin(q1R))/4503599627370496) + (7514214926474921*sin(q2R)*((3148506117433717*cos(q1R))/4503599627370496 + (1211728953682539*sin(q1R))/2251799813685248))/36893488147419103232) + (9007199067919185*cos(q3R)*((28359221366286827792295350160645*cos(q1R))/40564819207303340847894502572032 + (10914283902180054573281797610715*sin(q1R))/20282409603651670423947251286016 - 3983318308679801924058395430653/41538374868278621028243970633760768))/9007199254740992))/306499108173177771671669405430061836723747824436720435200000 - (608651409044468601*sin(q4R)*((7514214926474921*sin(q3R)*((4774755754024928798560446539205*cos(q2R))/10141204801825835211973625643008 + (7514214926474921*cos(q2R)*((3148506117433717*cos(q1R))/4503599627370496 + (1211728953682539*sin(q1R))/2251799813685248))/36893488147419103232 - sin(q2R)*((1211728953682539*cos(q1R))/2251799813685248 - (3148506117433717*sin(q1R))/4503599627370496)))/36893488147419103232 - cos(q3R)*((4774755754024928798560446539205*sin(q2R))/10141204801825835211973625643008 + cos(q2R)*((1211728953682539*cos(q1R))/2251799813685248 - (3148506117433717*sin(q1R))/4503599627370496) + (7514214926474921*sin(q2R)*((3148506117433717*cos(q1R))/4503599627370496 + (1211728953682539*sin(q1R))/2251799813685248))/36893488147419103232) + (9007199067919185*sin(q3R)*((28359221366286827792295350160645*cos(q1R))/40564819207303340847894502572032 + (10914283902180054573281797610715*sin(q1R))/20282409603651670423947251286016 - 3983318308679801924058395430653/41538374868278621028243970633760768))/9007199254740992))/73786976294838206464000 + (81*((7514214926474921*cos(q4R))/36893488147419103232 + (4503599440548691*sin(q4R))/4503599627370496)*((7514214926474921*cos(q3R)*((4774755754024928798560446539205*cos(q2R))/10141204801825835211973625643008 + (7514214926474921*cos(q2R)*((3148506117433717*cos(q1R))/4503599627370496 + (1211728953682539*sin(q1R))/2251799813685248))/36893488147419103232 - sin(q2R)*((1211728953682539*cos(q1R))/2251799813685248 - (3148506117433717*sin(q1R))/4503599627370496)))/36893488147419103232 + sin(q3R)*((4774755754024928798560446539205*sin(q2R))/10141204801825835211973625643008 + cos(q2R)*((1211728953682539*cos(q1R))/2251799813685248 - (3148506117433717*sin(q1R))/4503599627370496) + (7514214926474921*sin(q2R)*((3148506117433717*cos(q1R))/4503599627370496 + (1211728953682539*sin(q1R))/2251799813685248))/36893488147419103232) + (9007199067919185*cos(q3R)*((28359221366286827792295350160645*cos(q1R))/40564819207303340847894502572032 + (10914283902180054573281797610715*sin(q1R))/20282409603651670423947251286016 - 3983318308679801924058395430653/41538374868278621028243970633760768))/9007199254740992))/2000 - (712008244765680093343103025701132101054572137019*cos(q5R)*(((4503599440548691*cos(q4R))/4503599627370496 - (7514214926474921*sin(q4R))/36893488147419103232)*((7514214926474921*cos(q3R)*((4774755754024928798560446539205*cos(q2R))/10141204801825835211973625643008 + (7514214926474921*cos(q2R)*((3148506117433717*cos(q1R))/4503599627370496 + (1211728953682539*sin(q1R))/2251799813685248))/36893488147419103232 - sin(q2R)*((1211728953682539*cos(q1R))/2251799813685248 - (3148506117433717*sin(q1R))/4503599627370496)))/36893488147419103232 + sin(q3R)*((4774755754024928798560446539205*sin(q2R))/10141204801825835211973625643008 + cos(q2R)*((1211728953682539*cos(q1R))/2251799813685248 - (3148506117433717*sin(q1R))/4503599627370496) + (7514214926474921*sin(q2R)*((3148506117433717*cos(q1R))/4503599627370496 + (1211728953682539*sin(q1R))/2251799813685248))/36893488147419103232) + (9007199067919185*cos(q3R)*((28359221366286827792295350160645*cos(q1R))/40564819207303340847894502572032 + (10914283902180054573281797610715*sin(q1R))/20282409603651670423947251286016 - 3983318308679801924058395430653/41538374868278621028243970633760768))/9007199254740992) - (7514214926474921*cos(q4R)*((7514214926474921*sin(q3R)*((4774755754024928798560446539205*cos(q2R))/10141204801825835211973625643008 + (7514214926474921*cos(q2R)*((3148506117433717*cos(q1R))/4503599627370496 + (1211728953682539*sin(q1R))/2251799813685248))/36893488147419103232 - sin(q2R)*((1211728953682539*cos(q1R))/2251799813685248 - (3148506117433717*sin(q1R))/4503599627370496)))/36893488147419103232 - cos(q3R)*((4774755754024928798560446539205*sin(q2R))/10141204801825835211973625643008 + cos(q2R)*((1211728953682539*cos(q1R))/2251799813685248 - (3148506117433717*sin(q1R))/4503599627370496) + (7514214926474921*sin(q2R)*((3148506117433717*cos(q1R))/4503599627370496 + (1211728953682539*sin(q1R))/2251799813685248))/36893488147419103232) + (9007199067919185*sin(q3R)*((28359221366286827792295350160645*cos(q1R))/40564819207303340847894502572032 + (10914283902180054573281797610715*sin(q1R))/20282409603651670423947251286016 - 3983318308679801924058395430653/41538374868278621028243970633760768))/9007199254740992))/36893488147419103232))/2451992865385422173373355243440494693789982595493763481600 + (455490404115240510935077772268745492204390157443214084883134054419271951750419293234291596923751*cos(q3R)*((4774755754024928798560446539205*cos(q2R))/10141204801825835211973625643008 + (7514214926474921*cos(q2R)*((3148506117433717*cos(q1R))/4503599627370496 + (1211728953682539*sin(q1R))/2251799813685248))/36893488147419103232 - sin(q2R)*((1211728953682539*cos(q1R))/2251799813685248 - (3148506117433717*sin(q1R))/4503599627370496)))/53399675898022752059875542654238802865067613058916319248676040195555493144516013750574052173414400000 + (584133382113593486367040631332731*cos(q6R)*((9007199067919185*((4503599440548691*cos(q4R))/4503599627370496 - (7514214926474921*sin(q4R))/36893488147419103232)*((7514214926474921*cos(q3R)*((4774755754024928798560446539205*cos(q2R))/10141204801825835211973625643008 + (7514214926474921*cos(q2R)*((3148506117433717*cos(q1R))/4503599627370496 + (1211728953682539*sin(q1R))/2251799813685248))/36893488147419103232 - sin(q2R)*((1211728953682539*cos(q1R))/2251799813685248 - (3148506117433717*sin(q1R))/4503599627370496)))/36893488147419103232 + sin(q3R)*((4774755754024928798560446539205*sin(q2R))/10141204801825835211973625643008 + cos(q2R)*((1211728953682539*cos(q1R))/2251799813685248 - (3148506117433717*sin(q1R))/4503599627370496) + (7514214926474921*sin(q2R)*((3148506117433717*cos(q1R))/4503599627370496 + (1211728953682539*sin(q1R))/2251799813685248))/36893488147419103232) + (9007199067919185*cos(q3R)*((28359221366286827792295350160645*cos(q1R))/40564819207303340847894502572032 + (10914283902180054573281797610715*sin(q1R))/20282409603651670423947251286016 - 3983318308679801924058395430653/41538374868278621028243970633760768))/9007199254740992))/9007199254740992 + (13258697167433729449897784796786197386719169465*cos(q3R)*((4774755754024928798560446539205*cos(q2R))/10141204801825835211973625643008 + (7514214926474921*cos(q2R)*((3148506117433717*cos(q1R))/4503599627370496 + (1211728953682539*sin(q1R))/2251799813685248))/36893488147419103232 - sin(q2R)*((1211728953682539*cos(q1R))/2251799813685248 - (3148506117433717*sin(q1R))/4503599627370496)))/1569275433846670190958947355801916604025588861116008628224 - (67682029681889335677290557259385*cos(q3R)*((4774755754024928798560446539205*sin(q2R))/10141204801825835211973625643008 + cos(q2R)*((1211728953682539*cos(q1R))/2251799813685248 - (3148506117433717*sin(q1R))/4503599627370496) + (7514214926474921*sin(q2R)*((3148506117433717*cos(q1R))/4503599627370496 + (1211728953682539*sin(q1R))/2251799813685248))/36893488147419103232))/332306998946228968225951765070086144 + (508577317689771495245073589786522929324694383585*sin(q3R)*((4774755754024928798560446539205*cos(q2R))/10141204801825835211973625643008 + (7514214926474921*cos(q2R)*((3148506117433717*cos(q1R))/4503599627370496 + (1211728953682539*sin(q1R))/2251799813685248))/36893488147419103232 - sin(q2R)*((1211728953682539*cos(q1R))/2251799813685248 - (3148506117433717*sin(q1R))/4503599627370496)))/12259964326927110866866776217202473468949912977468817408 + (1764482024691522628700660907665*sin(q3R)*((4774755754024928798560446539205*sin(q2R))/10141204801825835211973625643008 + cos(q2R)*((1211728953682539*cos(q1R))/2251799813685248 - (3148506117433717*sin(q1R))/4503599627370496) + (7514214926474921*sin(q2R)*((3148506117433717*cos(q1R))/4503599627370496 + (1211728953682539*sin(q1R))/2251799813685248))/36893488147419103232))/42535295865117307932921825928971026432 + (15893040848161638993908057577265778144967053025*cos(q3R)*((28359221366286827792295350160645*cos(q1R))/40564819207303340847894502572032 + (10914283902180054573281797610715*sin(q1R))/20282409603651670423947251286016 - 3983318308679801924058395430653/41538374868278621028243970633760768))/383123885216472214589586756787577295904684780545900544 - (67682029681889335677290557259385*cos(q4R)*((7514214926474921*sin(q3R)*((4774755754024928798560446539205*cos(q2R))/10141204801825835211973625643008 + (7514214926474921*cos(q2R)*((3148506117433717*cos(q1R))/4503599627370496 + (1211728953682539*sin(q1R))/2251799813685248))/36893488147419103232 - sin(q2R)*((1211728953682539*cos(q1R))/2251799813685248 - (3148506117433717*sin(q1R))/4503599627370496)))/36893488147419103232 - cos(q3R)*((4774755754024928798560446539205*sin(q2R))/10141204801825835211973625643008 + cos(q2R)*((1211728953682539*cos(q1R))/2251799813685248 - (3148506117433717*sin(q1R))/4503599627370496) + (7514214926474921*sin(q2R)*((3148506117433717*cos(q1R))/4503599627370496 + (1211728953682539*sin(q1R))/2251799813685248))/36893488147419103232) + (9007199067919185*sin(q3R)*((28359221366286827792295350160645*cos(q1R))/40564819207303340847894502572032 + (10914283902180054573281797610715*sin(q1R))/20282409603651670423947251286016 - 3983318308679801924058395430653/41538374868278621028243970633760768))/9007199254740992))/332306998946228968225951765070086144 + (609625514665592237562888769449172969868262801225*sin(q3R)*((28359221366286827792295350160645*cos(q1R))/40564819207303340847894502572032 + (10914283902180054573281797610715*sin(q1R))/20282409603651670423947251286016 - 3983318308679801924058395430653/41538374868278621028243970633760768))/2993155353253689176481146537402947624255349848014848))/16225927682921336339157801028812800 + (202883803014822867*sin(q5R)*(((4503599440548691*cos(q4R))/4503599627370496 - (7514214926474921*sin(q4R))/36893488147419103232)*((7514214926474921*cos(q3R)*((4774755754024928798560446539205*cos(q2R))/10141204801825835211973625643008 + (7514214926474921*cos(q2R)*((3148506117433717*cos(q1R))/4503599627370496 + (1211728953682539*sin(q1R))/2251799813685248))/36893488147419103232 - sin(q2R)*((1211728953682539*cos(q1R))/2251799813685248 - (3148506117433717*sin(q1R))/4503599627370496)))/36893488147419103232 + sin(q3R)*((4774755754024928798560446539205*sin(q2R))/10141204801825835211973625643008 + cos(q2R)*((1211728953682539*cos(q1R))/2251799813685248 - (3148506117433717*sin(q1R))/4503599627370496) + (7514214926474921*sin(q2R)*((3148506117433717*cos(q1R))/4503599627370496 + (1211728953682539*sin(q1R))/2251799813685248))/36893488147419103232) + (9007199067919185*cos(q3R)*((28359221366286827792295350160645*cos(q1R))/40564819207303340847894502572032 + (10914283902180054573281797610715*sin(q1R))/20282409603651670423947251286016 - 3983318308679801924058395430653/41538374868278621028243970633760768))/9007199254740992) - (7514214926474921*cos(q4R)*((7514214926474921*sin(q3R)*((4774755754024928798560446539205*cos(q2R))/10141204801825835211973625643008 + (7514214926474921*cos(q2R)*((3148506117433717*cos(q1R))/4503599627370496 + (1211728953682539*sin(q1R))/2251799813685248))/36893488147419103232 - sin(q2R)*((1211728953682539*cos(q1R))/2251799813685248 - (3148506117433717*sin(q1R))/4503599627370496)))/36893488147419103232 - cos(q3R)*((4774755754024928798560446539205*sin(q2R))/10141204801825835211973625643008 + cos(q2R)*((1211728953682539*cos(q1R))/2251799813685248 - (3148506117433717*sin(q1R))/4503599627370496) + (7514214926474921*sin(q2R)*((3148506117433717*cos(q1R))/4503599627370496 + (1211728953682539*sin(q1R))/2251799813685248))/36893488147419103232) + (9007199067919185*sin(q3R)*((28359221366286827792295350160645*cos(q1R))/40564819207303340847894502572032 + (10914283902180054573281797610715*sin(q1R))/20282409603651670423947251286016 - 3983318308679801924058395430653/41538374868278621028243970633760768))/9007199254740992))/36893488147419103232))/36893488147419103232000 + (27*cos(q5R)*((7514214926474921*sin(q4R)*((7514214926474921*sin(q3R)*((4774755754024928798560446539205*cos(q2R))/10141204801825835211973625643008 + (7514214926474921*cos(q2R)*((3148506117433717*cos(q1R))/4503599627370496 + (1211728953682539*sin(q1R))/2251799813685248))/36893488147419103232 - sin(q2R)*((1211728953682539*cos(q1R))/2251799813685248 - (3148506117433717*sin(q1R))/4503599627370496)))/36893488147419103232 - cos(q3R)*((4774755754024928798560446539205*sin(q2R))/10141204801825835211973625643008 + cos(q2R)*((1211728953682539*cos(q1R))/2251799813685248 - (3148506117433717*sin(q1R))/4503599627370496) + (7514214926474921*sin(q2R)*((3148506117433717*cos(q1R))/4503599627370496 + (1211728953682539*sin(q1R))/2251799813685248))/36893488147419103232) + (9007199067919185*sin(q3R)*((28359221366286827792295350160645*cos(q1R))/40564819207303340847894502572032 + (10914283902180054573281797610715*sin(q1R))/20282409603651670423947251286016 - 3983318308679801924058395430653/41538374868278621028243970633760768))/9007199254740992))/36893488147419103232 - ((7514214926474921*cos(q4R))/36893488147419103232 + (4503599440548691*sin(q4R))/4503599627370496)*((7514214926474921*cos(q3R)*((4774755754024928798560446539205*cos(q2R))/10141204801825835211973625643008 + (7514214926474921*cos(q2R)*((3148506117433717*cos(q1R))/4503599627370496 + (1211728953682539*sin(q1R))/2251799813685248))/36893488147419103232 - sin(q2R)*((1211728953682539*cos(q1R))/2251799813685248 - (3148506117433717*sin(q1R))/4503599627370496)))/36893488147419103232 + sin(q3R)*((4774755754024928798560446539205*sin(q2R))/10141204801825835211973625643008 + cos(q2R)*((1211728953682539*cos(q1R))/2251799813685248 - (3148506117433717*sin(q1R))/4503599627370496) + (7514214926474921*sin(q2R)*((3148506117433717*cos(q1R))/4503599627370496 + (1211728953682539*sin(q1R))/2251799813685248))/36893488147419103232) + (9007199067919185*cos(q3R)*((28359221366286827792295350160645*cos(q1R))/40564819207303340847894502572032 + (10914283902180054573281797610715*sin(q1R))/20282409603651670423947251286016 - 3983318308679801924058395430653/41538374868278621028243970633760768))/9007199254740992)))/1000 - (46241644459901303158631016767207157814229090534989303509431886332469146043*cos(q3R)*((4774755754024928798560446539205*sin(q2R))/10141204801825835211973625643008 + cos(q2R)*((1211728953682539*cos(q1R))/2251799813685248 - (3148506117433717*sin(q1R))/4503599627370496) + (7514214926474921*sin(q2R)*((3148506117433717*cos(q1R))/4503599627370496 + (1211728953682539*sin(q1R))/2251799813685248))/36893488147419103232))/2261564242916331941866620800950935700259179388000792266395655937654553313280000 + (347469655025336708709976918716104493695816557877713443586884917071777956519687017125887603*sin(q3R)*((4774755754024928798560446539205*cos(q2R))/10141204801825835211973625643008 + (7514214926474921*cos(q2R)*((3148506117433717*cos(q1R))/4503599627370496 + (1211728953682539*sin(q1R))/2251799813685248))/36893488147419103232 - sin(q2R)*((1211728953682539*cos(q1R))/2251799813685248 - (3148506117433717*sin(q1R))/4503599627370496)))/83436993590660550093555535397248129476668145404556748826056312805555458038306271485271956520960000 + (48638874966763599*sin(q6R)*((9007199067919185*((4503599440548691*cos(q4R))/4503599627370496 - (7514214926474921*sin(q4R))/36893488147419103232)*((7514214926474921*cos(q3R)*((4774755754024928798560446539205*cos(q2R))/10141204801825835211973625643008 + (7514214926474921*cos(q2R)*((3148506117433717*cos(q1R))/4503599627370496 + (1211728953682539*sin(q1R))/2251799813685248))/36893488147419103232 - sin(q2R)*((1211728953682539*cos(q1R))/2251799813685248 - (3148506117433717*sin(q1R))/4503599627370496)))/36893488147419103232 + sin(q3R)*((4774755754024928798560446539205*sin(q2R))/10141204801825835211973625643008 + cos(q2R)*((1211728953682539*cos(q1R))/2251799813685248 - (3148506117433717*sin(q1R))/4503599627370496) + (7514214926474921*sin(q2R)*((3148506117433717*cos(q1R))/4503599627370496 + (1211728953682539*sin(q1R))/2251799813685248))/36893488147419103232) + (9007199067919185*cos(q3R)*((28359221366286827792295350160645*cos(q1R))/40564819207303340847894502572032 + (10914283902180054573281797610715*sin(q1R))/20282409603651670423947251286016 - 3983318308679801924058395430653/41538374868278621028243970633760768))/9007199254740992))/9007199254740992 + (13258697167433729449897784796786197386719169465*cos(q3R)*((4774755754024928798560446539205*cos(q2R))/10141204801825835211973625643008 + (7514214926474921*cos(q2R)*((3148506117433717*cos(q1R))/4503599627370496 + (1211728953682539*sin(q1R))/2251799813685248))/36893488147419103232 - sin(q2R)*((1211728953682539*cos(q1R))/2251799813685248 - (3148506117433717*sin(q1R))/4503599627370496)))/1569275433846670190958947355801916604025588861116008628224 - (67682029681889335677290557259385*cos(q3R)*((4774755754024928798560446539205*sin(q2R))/10141204801825835211973625643008 + cos(q2R)*((1211728953682539*cos(q1R))/2251799813685248 - (3148506117433717*sin(q1R))/4503599627370496) + (7514214926474921*sin(q2R)*((3148506117433717*cos(q1R))/4503599627370496 + (1211728953682539*sin(q1R))/2251799813685248))/36893488147419103232))/332306998946228968225951765070086144 + (508577317689771495245073589786522929324694383585*sin(q3R)*((4774755754024928798560446539205*cos(q2R))/10141204801825835211973625643008 + (7514214926474921*cos(q2R)*((3148506117433717*cos(q1R))/4503599627370496 + (1211728953682539*sin(q1R))/2251799813685248))/36893488147419103232 - sin(q2R)*((1211728953682539*cos(q1R))/2251799813685248 - (3148506117433717*sin(q1R))/4503599627370496)))/12259964326927110866866776217202473468949912977468817408 + (1764482024691522628700660907665*sin(q3R)*((4774755754024928798560446539205*sin(q2R))/10141204801825835211973625643008 + cos(q2R)*((1211728953682539*cos(q1R))/2251799813685248 - (3148506117433717*sin(q1R))/4503599627370496) + (7514214926474921*sin(q2R)*((3148506117433717*cos(q1R))/4503599627370496 + (1211728953682539*sin(q1R))/2251799813685248))/36893488147419103232))/42535295865117307932921825928971026432 + (15893040848161638993908057577265778144967053025*cos(q3R)*((28359221366286827792295350160645*cos(q1R))/40564819207303340847894502572032 + (10914283902180054573281797610715*sin(q1R))/20282409603651670423947251286016 - 3983318308679801924058395430653/41538374868278621028243970633760768))/383123885216472214589586756787577295904684780545900544 - (67682029681889335677290557259385*cos(q4R)*((7514214926474921*sin(q3R)*((4774755754024928798560446539205*cos(q2R))/10141204801825835211973625643008 + (7514214926474921*cos(q2R)*((3148506117433717*cos(q1R))/4503599627370496 + (1211728953682539*sin(q1R))/2251799813685248))/36893488147419103232 - sin(q2R)*((1211728953682539*cos(q1R))/2251799813685248 - (3148506117433717*sin(q1R))/4503599627370496)))/36893488147419103232 - cos(q3R)*((4774755754024928798560446539205*sin(q2R))/10141204801825835211973625643008 + cos(q2R)*((1211728953682539*cos(q1R))/2251799813685248 - (3148506117433717*sin(q1R))/4503599627370496) + (7514214926474921*sin(q2R)*((3148506117433717*cos(q1R))/4503599627370496 + (1211728953682539*sin(q1R))/2251799813685248))/36893488147419103232) + (9007199067919185*sin(q3R)*((28359221366286827792295350160645*cos(q1R))/40564819207303340847894502572032 + (10914283902180054573281797610715*sin(q1R))/20282409603651670423947251286016 - 3983318308679801924058395430653/41538374868278621028243970633760768))/9007199254740992))/332306998946228968225951765070086144 + (609625514665592237562888769449172969868262801225*sin(q3R)*((28359221366286827792295350160645*cos(q1R))/40564819207303340847894502572032 + (10914283902180054573281797610715*sin(q1R))/20282409603651670423947251286016 - 3983318308679801924058395430653/41538374868278621028243970633760768))/2993155353253689176481146537402947624255349848014848))/1801439850948198400 + (94754841554645069948206780163139*sin(q5R)*((7514214926474921*sin(q4R)*((7514214926474921*sin(q3R)*((4774755754024928798560446539205*cos(q2R))/10141204801825835211973625643008 + (7514214926474921*cos(q2R)*((3148506117433717*cos(q1R))/4503599627370496 + (1211728953682539*sin(q1R))/2251799813685248))/36893488147419103232 - sin(q2R)*((1211728953682539*cos(q1R))/2251799813685248 - (3148506117433717*sin(q1R))/4503599627370496)))/36893488147419103232 - cos(q3R)*((4774755754024928798560446539205*sin(q2R))/10141204801825835211973625643008 + cos(q2R)*((1211728953682539*cos(q1R))/2251799813685248 - (3148506117433717*sin(q1R))/4503599627370496) + (7514214926474921*sin(q2R)*((3148506117433717*cos(q1R))/4503599627370496 + (1211728953682539*sin(q1R))/2251799813685248))/36893488147419103232) + (9007199067919185*sin(q3R)*((28359221366286827792295350160645*cos(q1R))/40564819207303340847894502572032 + (10914283902180054573281797610715*sin(q1R))/20282409603651670423947251286016 - 3983318308679801924058395430653/41538374868278621028243970633760768))/9007199254740992))/36893488147419103232 - ((7514214926474921*cos(q4R))/36893488147419103232 + (4503599440548691*sin(q4R))/4503599627370496)*((7514214926474921*cos(q3R)*((4774755754024928798560446539205*cos(q2R))/10141204801825835211973625643008 + (7514214926474921*cos(q2R)*((3148506117433717*cos(q1R))/4503599627370496 + (1211728953682539*sin(q1R))/2251799813685248))/36893488147419103232 - sin(q2R)*((1211728953682539*cos(q1R))/2251799813685248 - (3148506117433717*sin(q1R))/4503599627370496)))/36893488147419103232 + sin(q3R)*((4774755754024928798560446539205*sin(q2R))/10141204801825835211973625643008 + cos(q2R)*((1211728953682539*cos(q1R))/2251799813685248 - (3148506117433717*sin(q1R))/4503599627370496) + (7514214926474921*sin(q2R)*((3148506117433717*cos(q1R))/4503599627370496 + (1211728953682539*sin(q1R))/2251799813685248))/36893488147419103232) + (9007199067919185*cos(q3R)*((28359221366286827792295350160645*cos(q1R))/40564819207303340847894502572032 + (10914283902180054573281797610715*sin(q1R))/20282409603651670423947251286016 - 3983318308679801924058395430653/41538374868278621028243970633760768))/9007199254740992)))/66461399789245793645190353014017228800 + (60617164743372705924380750591060836759586313939367162716784907429017787816377231*sin(q3R)*((4774755754024928798560446539205*sin(q2R))/10141204801825835211973625643008 + cos(q2R)*((1211728953682539*cos(q1R))/2251799813685248 - (3148506117433717*sin(q1R))/4503599627370496) + (7514214926474921*sin(q2R)*((3148506117433717*cos(q1R))/4503599627370496 + (1211728953682539*sin(q1R))/2251799813685248))/36893488147419103232))/1447401115466452442794637312608598848165874808320507050493219800098914120499200000 - (2436553109258773196144549622003023*cos(q6R)*(sin(q5R)*((7514214926474921*sin(q4R)*((7514214926474921*sin(q3R)*((4774755754024928798560446539205*cos(q2R))/10141204801825835211973625643008 + (7514214926474921*cos(q2R)*((3148506117433717*cos(q1R))/4503599627370496 + (1211728953682539*sin(q1R))/2251799813685248))/36893488147419103232 - sin(q2R)*((1211728953682539*cos(q1R))/2251799813685248 - (3148506117433717*sin(q1R))/4503599627370496)))/36893488147419103232 - cos(q3R)*((4774755754024928798560446539205*sin(q2R))/10141204801825835211973625643008 + cos(q2R)*((1211728953682539*cos(q1R))/2251799813685248 - (3148506117433717*sin(q1R))/4503599627370496) + (7514214926474921*sin(q2R)*((3148506117433717*cos(q1R))/4503599627370496 + (1211728953682539*sin(q1R))/2251799813685248))/36893488147419103232) + (9007199067919185*sin(q3R)*((28359221366286827792295350160645*cos(q1R))/40564819207303340847894502572032 + (10914283902180054573281797610715*sin(q1R))/20282409603651670423947251286016 - 3983318308679801924058395430653/41538374868278621028243970633760768))/9007199254740992))/36893488147419103232 - ((7514214926474921*cos(q4R))/36893488147419103232 + (4503599440548691*sin(q4R))/4503599627370496)*((7514214926474921*cos(q3R)*((4774755754024928798560446539205*cos(q2R))/10141204801825835211973625643008 + (7514214926474921*cos(q2R)*((3148506117433717*cos(q1R))/4503599627370496 + (1211728953682539*sin(q1R))/2251799813685248))/36893488147419103232 - sin(q2R)*((1211728953682539*cos(q1R))/2251799813685248 - (3148506117433717*sin(q1R))/4503599627370496)))/36893488147419103232 + sin(q3R)*((4774755754024928798560446539205*sin(q2R))/10141204801825835211973625643008 + cos(q2R)*((1211728953682539*cos(q1R))/2251799813685248 - (3148506117433717*sin(q1R))/4503599627370496) + (7514214926474921*sin(q2R)*((3148506117433717*cos(q1R))/4503599627370496 + (1211728953682539*sin(q1R))/2251799813685248))/36893488147419103232) + (9007199067919185*cos(q3R)*((28359221366286827792295350160645*cos(q1R))/40564819207303340847894502572032 + (10914283902180054573281797610715*sin(q1R))/20282409603651670423947251286016 - 3983318308679801924058395430653/41538374868278621028243970633760768))/9007199254740992)) - (7514214926474921*cos(q5R)*(((4503599440548691*cos(q4R))/4503599627370496 - (7514214926474921*sin(q4R))/36893488147419103232)*((7514214926474921*cos(q3R)*((4774755754024928798560446539205*cos(q2R))/10141204801825835211973625643008 + (7514214926474921*cos(q2R)*((3148506117433717*cos(q1R))/4503599627370496 + (1211728953682539*sin(q1R))/2251799813685248))/36893488147419103232 - sin(q2R)*((1211728953682539*cos(q1R))/2251799813685248 - (3148506117433717*sin(q1R))/4503599627370496)))/36893488147419103232 + sin(q3R)*((4774755754024928798560446539205*sin(q2R))/10141204801825835211973625643008 + cos(q2R)*((1211728953682539*cos(q1R))/2251799813685248 - (3148506117433717*sin(q1R))/4503599627370496) + (7514214926474921*sin(q2R)*((3148506117433717*cos(q1R))/4503599627370496 + (1211728953682539*sin(q1R))/2251799813685248))/36893488147419103232) + (9007199067919185*cos(q3R)*((28359221366286827792295350160645*cos(q1R))/40564819207303340847894502572032 + (10914283902180054573281797610715*sin(q1R))/20282409603651670423947251286016 - 3983318308679801924058395430653/41538374868278621028243970633760768))/9007199254740992) - (7514214926474921*cos(q4R)*((7514214926474921*sin(q3R)*((4774755754024928798560446539205*cos(q2R))/10141204801825835211973625643008 + (7514214926474921*cos(q2R)*((3148506117433717*cos(q1R))/4503599627370496 + (1211728953682539*sin(q1R))/2251799813685248))/36893488147419103232 - sin(q2R)*((1211728953682539*cos(q1R))/2251799813685248 - (3148506117433717*sin(q1R))/4503599627370496)))/36893488147419103232 - cos(q3R)*((4774755754024928798560446539205*sin(q2R))/10141204801825835211973625643008 + cos(q2R)*((1211728953682539*cos(q1R))/2251799813685248 - (3148506117433717*sin(q1R))/4503599627370496) + (7514214926474921*sin(q2R)*((3148506117433717*cos(q1R))/4503599627370496 + (1211728953682539*sin(q1R))/2251799813685248))/36893488147419103232) + (9007199067919185*sin(q3R)*((28359221366286827792295350160645*cos(q1R))/40564819207303340847894502572032 + (10914283902180054573281797610715*sin(q1R))/20282409603651670423947251286016 - 3983318308679801924058395430653/41538374868278621028243970633760768))/9007199254740992))/36893488147419103232))/36893488147419103232 + (9007199067919185*cos(q5R)*((1764482024691522628700660907665*cos(q3R)*((4774755754024928798560446539205*cos(q2R))/10141204801825835211973625643008 + (7514214926474921*cos(q2R)*((3148506117433717*cos(q1R))/4503599627370496 + (1211728953682539*sin(q1R))/2251799813685248))/36893488147419103232 - sin(q2R)*((1211728953682539*cos(q1R))/2251799813685248 - (3148506117433717*sin(q1R))/4503599627370496)))/42535295865117307932921825928971026432 - (9007199067919185*cos(q3R)*((4774755754024928798560446539205*sin(q2R))/10141204801825835211973625643008 + cos(q2R)*((1211728953682539*cos(q1R))/2251799813685248 - (3148506117433717*sin(q1R))/4503599627370496) + (7514214926474921*sin(q2R)*((3148506117433717*cos(q1R))/4503599627370496 + (1211728953682539*sin(q1R))/2251799813685248))/36893488147419103232))/9007199254740992 + (67682029681889335677290557259385*sin(q3R)*((4774755754024928798560446539205*cos(q2R))/10141204801825835211973625643008 + (7514214926474921*cos(q2R)*((3148506117433717*cos(q1R))/4503599627370496 + (1211728953682539*sin(q1R))/2251799813685248))/36893488147419103232 - sin(q2R)*((1211728953682539*cos(q1R))/2251799813685248 - (3148506117433717*sin(q1R))/4503599627370496)))/332306998946228968225951765070086144 + (234819211581865*sin(q3R)*((4774755754024928798560446539205*sin(q2R))/10141204801825835211973625643008 + cos(q2R)*((1211728953682539*cos(q1R))/2251799813685248 - (3148506117433717*sin(q1R))/4503599627370496) + (7514214926474921*sin(q2R)*((3148506117433717*cos(q1R))/4503599627370496 + (1211728953682539*sin(q1R))/2251799813685248))/36893488147419103232))/1152921504606846976 + (2115063383689692319117831580025*cos(q3R)*((28359221366286827792295350160645*cos(q1R))/40564819207303340847894502572032 + (10914283902180054573281797610715*sin(q1R))/20282409603651670423947251286016 - 3983318308679801924058395430653/41538374868278621028243970633760768))/10384593717069655257060992658440192 + (81129635049124235038645691064225*sin(q3R)*((28359221366286827792295350160645*cos(q1R))/40564819207303340847894502572032 + (10914283902180054573281797610715*sin(q1R))/20282409603651670423947251286016 - 3983318308679801924058395430653/41538374868278621028243970633760768))/81129638414606681695789005144064))/9007199254740992))/332306998946228968225951765070086144000 - (27*cos(q6R)*((7514214926474921*sin(q5R)*(((4503599440548691*cos(q4R))/4503599627370496 - (7514214926474921*sin(q4R))/36893488147419103232)*((7514214926474921*cos(q3R)*((4774755754024928798560446539205*cos(q2R))/10141204801825835211973625643008 + (7514214926474921*cos(q2R)*((3148506117433717*cos(q1R))/4503599627370496 + (1211728953682539*sin(q1R))/2251799813685248))/36893488147419103232 - sin(q2R)*((1211728953682539*cos(q1R))/2251799813685248 - (3148506117433717*sin(q1R))/4503599627370496)))/36893488147419103232 + sin(q3R)*((4774755754024928798560446539205*sin(q2R))/10141204801825835211973625643008 + cos(q2R)*((1211728953682539*cos(q1R))/2251799813685248 - (3148506117433717*sin(q1R))/4503599627370496) + (7514214926474921*sin(q2R)*((3148506117433717*cos(q1R))/4503599627370496 + (1211728953682539*sin(q1R))/2251799813685248))/36893488147419103232) + (9007199067919185*cos(q3R)*((28359221366286827792295350160645*cos(q1R))/40564819207303340847894502572032 + (10914283902180054573281797610715*sin(q1R))/20282409603651670423947251286016 - 3983318308679801924058395430653/41538374868278621028243970633760768))/9007199254740992) - (7514214926474921*cos(q4R)*((7514214926474921*sin(q3R)*((4774755754024928798560446539205*cos(q2R))/10141204801825835211973625643008 + (7514214926474921*cos(q2R)*((3148506117433717*cos(q1R))/4503599627370496 + (1211728953682539*sin(q1R))/2251799813685248))/36893488147419103232 - sin(q2R)*((1211728953682539*cos(q1R))/2251799813685248 - (3148506117433717*sin(q1R))/4503599627370496)))/36893488147419103232 - cos(q3R)*((4774755754024928798560446539205*sin(q2R))/10141204801825835211973625643008 + cos(q2R)*((1211728953682539*cos(q1R))/2251799813685248 - (3148506117433717*sin(q1R))/4503599627370496) + (7514214926474921*sin(q2R)*((3148506117433717*cos(q1R))/4503599627370496 + (1211728953682539*sin(q1R))/2251799813685248))/36893488147419103232) + (9007199067919185*sin(q3R)*((28359221366286827792295350160645*cos(q1R))/40564819207303340847894502572032 + (10914283902180054573281797610715*sin(q1R))/20282409603651670423947251286016 - 3983318308679801924058395430653/41538374868278621028243970633760768))/9007199254740992))/36893488147419103232))/36893488147419103232 + cos(q5R)*((7514214926474921*sin(q4R)*((7514214926474921*sin(q3R)*((4774755754024928798560446539205*cos(q2R))/10141204801825835211973625643008 + (7514214926474921*cos(q2R)*((3148506117433717*cos(q1R))/4503599627370496 + (1211728953682539*sin(q1R))/2251799813685248))/36893488147419103232 - sin(q2R)*((1211728953682539*cos(q1R))/2251799813685248 - (3148506117433717*sin(q1R))/4503599627370496)))/36893488147419103232 - cos(q3R)*((4774755754024928798560446539205*sin(q2R))/10141204801825835211973625643008 + cos(q2R)*((1211728953682539*cos(q1R))/2251799813685248 - (3148506117433717*sin(q1R))/4503599627370496) + (7514214926474921*sin(q2R)*((3148506117433717*cos(q1R))/4503599627370496 + (1211728953682539*sin(q1R))/2251799813685248))/36893488147419103232) + (9007199067919185*sin(q3R)*((28359221366286827792295350160645*cos(q1R))/40564819207303340847894502572032 + (10914283902180054573281797610715*sin(q1R))/20282409603651670423947251286016 - 3983318308679801924058395430653/41538374868278621028243970633760768))/9007199254740992))/36893488147419103232 - ((7514214926474921*cos(q4R))/36893488147419103232 + (4503599440548691*sin(q4R))/4503599627370496)*((7514214926474921*cos(q3R)*((4774755754024928798560446539205*cos(q2R))/10141204801825835211973625643008 + (7514214926474921*cos(q2R)*((3148506117433717*cos(q1R))/4503599627370496 + (1211728953682539*sin(q1R))/2251799813685248))/36893488147419103232 - sin(q2R)*((1211728953682539*cos(q1R))/2251799813685248 - (3148506117433717*sin(q1R))/4503599627370496)))/36893488147419103232 + sin(q3R)*((4774755754024928798560446539205*sin(q2R))/10141204801825835211973625643008 + cos(q2R)*((1211728953682539*cos(q1R))/2251799813685248 - (3148506117433717*sin(q1R))/4503599627370496) + (7514214926474921*sin(q2R)*((3148506117433717*cos(q1R))/4503599627370496 + (1211728953682539*sin(q1R))/2251799813685248))/36893488147419103232) + (9007199067919185*cos(q3R)*((28359221366286827792295350160645*cos(q1R))/40564819207303340847894502572032 + (10914283902180054573281797610715*sin(q1R))/20282409603651670423947251286016 - 3983318308679801924058395430653/41538374868278621028243970633760768))/9007199254740992)) - (9007199067919185*sin(q5R)*((1764482024691522628700660907665*cos(q3R)*((4774755754024928798560446539205*cos(q2R))/10141204801825835211973625643008 + (7514214926474921*cos(q2R)*((3148506117433717*cos(q1R))/4503599627370496 + (1211728953682539*sin(q1R))/2251799813685248))/36893488147419103232 - sin(q2R)*((1211728953682539*cos(q1R))/2251799813685248 - (3148506117433717*sin(q1R))/4503599627370496)))/42535295865117307932921825928971026432 - (9007199067919185*cos(q3R)*((4774755754024928798560446539205*sin(q2R))/10141204801825835211973625643008 + cos(q2R)*((1211728953682539*cos(q1R))/2251799813685248 - (3148506117433717*sin(q1R))/4503599627370496) + (7514214926474921*sin(q2R)*((3148506117433717*cos(q1R))/4503599627370496 + (1211728953682539*sin(q1R))/2251799813685248))/36893488147419103232))/9007199254740992 + (67682029681889335677290557259385*sin(q3R)*((4774755754024928798560446539205*cos(q2R))/10141204801825835211973625643008 + (7514214926474921*cos(q2R)*((3148506117433717*cos(q1R))/4503599627370496 + (1211728953682539*sin(q1R))/2251799813685248))/36893488147419103232 - sin(q2R)*((1211728953682539*cos(q1R))/2251799813685248 - (3148506117433717*sin(q1R))/4503599627370496)))/332306998946228968225951765070086144 + (234819211581865*sin(q3R)*((4774755754024928798560446539205*sin(q2R))/10141204801825835211973625643008 + cos(q2R)*((1211728953682539*cos(q1R))/2251799813685248 - (3148506117433717*sin(q1R))/4503599627370496) + (7514214926474921*sin(q2R)*((3148506117433717*cos(q1R))/4503599627370496 + (1211728953682539*sin(q1R))/2251799813685248))/36893488147419103232))/1152921504606846976 + (2115063383689692319117831580025*cos(q3R)*((28359221366286827792295350160645*cos(q1R))/40564819207303340847894502572032 + (10914283902180054573281797610715*sin(q1R))/20282409603651670423947251286016 - 3983318308679801924058395430653/41538374868278621028243970633760768))/10384593717069655257060992658440192 + (81129635049124235038645691064225*sin(q3R)*((28359221366286827792295350160645*cos(q1R))/40564819207303340847894502572032 + (10914283902180054573281797610715*sin(q1R))/20282409603651670423947251286016 - 3983318308679801924058395430653/41538374868278621028243970633760768))/81129638414606681695789005144064))/9007199254740992))/1000 - (202883803014822867*sin(q6R)*(sin(q5R)*((7514214926474921*sin(q4R)*((7514214926474921*sin(q3R)*((4774755754024928798560446539205*cos(q2R))/10141204801825835211973625643008 + (7514214926474921*cos(q2R)*((3148506117433717*cos(q1R))/4503599627370496 + (1211728953682539*sin(q1R))/2251799813685248))/36893488147419103232 - sin(q2R)*((1211728953682539*cos(q1R))/2251799813685248 - (3148506117433717*sin(q1R))/4503599627370496)))/36893488147419103232 - cos(q3R)*((4774755754024928798560446539205*sin(q2R))/10141204801825835211973625643008 + cos(q2R)*((1211728953682539*cos(q1R))/2251799813685248 - (3148506117433717*sin(q1R))/4503599627370496) + (7514214926474921*sin(q2R)*((3148506117433717*cos(q1R))/4503599627370496 + (1211728953682539*sin(q1R))/2251799813685248))/36893488147419103232) + (9007199067919185*sin(q3R)*((28359221366286827792295350160645*cos(q1R))/40564819207303340847894502572032 + (10914283902180054573281797610715*sin(q1R))/20282409603651670423947251286016 - 3983318308679801924058395430653/41538374868278621028243970633760768))/9007199254740992))/36893488147419103232 - ((7514214926474921*cos(q4R))/36893488147419103232 + (4503599440548691*sin(q4R))/4503599627370496)*((7514214926474921*cos(q3R)*((4774755754024928798560446539205*cos(q2R))/10141204801825835211973625643008 + (7514214926474921*cos(q2R)*((3148506117433717*cos(q1R))/4503599627370496 + (1211728953682539*sin(q1R))/2251799813685248))/36893488147419103232 - sin(q2R)*((1211728953682539*cos(q1R))/2251799813685248 - (3148506117433717*sin(q1R))/4503599627370496)))/36893488147419103232 + sin(q3R)*((4774755754024928798560446539205*sin(q2R))/10141204801825835211973625643008 + cos(q2R)*((1211728953682539*cos(q1R))/2251799813685248 - (3148506117433717*sin(q1R))/4503599627370496) + (7514214926474921*sin(q2R)*((3148506117433717*cos(q1R))/4503599627370496 + (1211728953682539*sin(q1R))/2251799813685248))/36893488147419103232) + (9007199067919185*cos(q3R)*((28359221366286827792295350160645*cos(q1R))/40564819207303340847894502572032 + (10914283902180054573281797610715*sin(q1R))/20282409603651670423947251286016 - 3983318308679801924058395430653/41538374868278621028243970633760768))/9007199254740992)) - (7514214926474921*cos(q5R)*(((4503599440548691*cos(q4R))/4503599627370496 - (7514214926474921*sin(q4R))/36893488147419103232)*((7514214926474921*cos(q3R)*((4774755754024928798560446539205*cos(q2R))/10141204801825835211973625643008 + (7514214926474921*cos(q2R)*((3148506117433717*cos(q1R))/4503599627370496 + (1211728953682539*sin(q1R))/2251799813685248))/36893488147419103232 - sin(q2R)*((1211728953682539*cos(q1R))/2251799813685248 - (3148506117433717*sin(q1R))/4503599627370496)))/36893488147419103232 + sin(q3R)*((4774755754024928798560446539205*sin(q2R))/10141204801825835211973625643008 + cos(q2R)*((1211728953682539*cos(q1R))/2251799813685248 - (3148506117433717*sin(q1R))/4503599627370496) + (7514214926474921*sin(q2R)*((3148506117433717*cos(q1R))/4503599627370496 + (1211728953682539*sin(q1R))/2251799813685248))/36893488147419103232) + (9007199067919185*cos(q3R)*((28359221366286827792295350160645*cos(q1R))/40564819207303340847894502572032 + (10914283902180054573281797610715*sin(q1R))/20282409603651670423947251286016 - 3983318308679801924058395430653/41538374868278621028243970633760768))/9007199254740992) - (7514214926474921*cos(q4R)*((7514214926474921*sin(q3R)*((4774755754024928798560446539205*cos(q2R))/10141204801825835211973625643008 + (7514214926474921*cos(q2R)*((3148506117433717*cos(q1R))/4503599627370496 + (1211728953682539*sin(q1R))/2251799813685248))/36893488147419103232 - sin(q2R)*((1211728953682539*cos(q1R))/2251799813685248 - (3148506117433717*sin(q1R))/4503599627370496)))/36893488147419103232 - cos(q3R)*((4774755754024928798560446539205*sin(q2R))/10141204801825835211973625643008 + cos(q2R)*((1211728953682539*cos(q1R))/2251799813685248 - (3148506117433717*sin(q1R))/4503599627370496) + (7514214926474921*sin(q2R)*((3148506117433717*cos(q1R))/4503599627370496 + (1211728953682539*sin(q1R))/2251799813685248))/36893488147419103232) + (9007199067919185*sin(q3R)*((28359221366286827792295350160645*cos(q1R))/40564819207303340847894502572032 + (10914283902180054573281797610715*sin(q1R))/20282409603651670423947251286016 - 3983318308679801924058395430653/41538374868278621028243970633760768))/9007199254740992))/36893488147419103232))/36893488147419103232 + (9007199067919185*cos(q5R)*((1764482024691522628700660907665*cos(q3R)*((4774755754024928798560446539205*cos(q2R))/10141204801825835211973625643008 + (7514214926474921*cos(q2R)*((3148506117433717*cos(q1R))/4503599627370496 + (1211728953682539*sin(q1R))/2251799813685248))/36893488147419103232 - sin(q2R)*((1211728953682539*cos(q1R))/2251799813685248 - (3148506117433717*sin(q1R))/4503599627370496)))/42535295865117307932921825928971026432 - (9007199067919185*cos(q3R)*((4774755754024928798560446539205*sin(q2R))/10141204801825835211973625643008 + cos(q2R)*((1211728953682539*cos(q1R))/2251799813685248 - (3148506117433717*sin(q1R))/4503599627370496) + (7514214926474921*sin(q2R)*((3148506117433717*cos(q1R))/4503599627370496 + (1211728953682539*sin(q1R))/2251799813685248))/36893488147419103232))/9007199254740992 + (67682029681889335677290557259385*sin(q3R)*((4774755754024928798560446539205*cos(q2R))/10141204801825835211973625643008 + (7514214926474921*cos(q2R)*((3148506117433717*cos(q1R))/4503599627370496 + (1211728953682539*sin(q1R))/2251799813685248))/36893488147419103232 - sin(q2R)*((1211728953682539*cos(q1R))/2251799813685248 - (3148506117433717*sin(q1R))/4503599627370496)))/332306998946228968225951765070086144 + (234819211581865*sin(q3R)*((4774755754024928798560446539205*sin(q2R))/10141204801825835211973625643008 + cos(q2R)*((1211728953682539*cos(q1R))/2251799813685248 - (3148506117433717*sin(q1R))/4503599627370496) + (7514214926474921*sin(q2R)*((3148506117433717*cos(q1R))/4503599627370496 + (1211728953682539*sin(q1R))/2251799813685248))/36893488147419103232))/1152921504606846976 + (2115063383689692319117831580025*cos(q3R)*((28359221366286827792295350160645*cos(q1R))/40564819207303340847894502572032 + (10914283902180054573281797610715*sin(q1R))/20282409603651670423947251286016 - 3983318308679801924058395430653/41538374868278621028243970633760768))/10384593717069655257060992658440192 + (81129635049124235038645691064225*sin(q3R)*((28359221366286827792295350160645*cos(q1R))/40564819207303340847894502572032 + (10914283902180054573281797610715*sin(q1R))/20282409603651670423947251286016 - 3983318308679801924058395430653/41538374868278621028243970633760768))/81129638414606681695789005144064))/9007199254740992))/36893488147419103232000 + (109198173955282063961996941994332957526645881091499469714283881779231664456243735535448036415347*cos(q3R)*((28359221366286827792295350160645*cos(q1R))/40564819207303340847894502572032 + (10914283902180054573281797610715*sin(q1R))/20282409603651670423947251286016 - 3983318308679801924058395430653/41538374868278621028243970633760768))/2607406049708142190423610481164004046145879543892398400814259775173608063697070983914748641280000 + (170695144106365826517608855445768431563113584343*cos(q5R)*((1764482024691522628700660907665*cos(q3R)*((4774755754024928798560446539205*cos(q2R))/10141204801825835211973625643008 + (7514214926474921*cos(q2R)*((3148506117433717*cos(q1R))/4503599627370496 + (1211728953682539*sin(q1R))/2251799813685248))/36893488147419103232 - sin(q2R)*((1211728953682539*cos(q1R))/2251799813685248 - (3148506117433717*sin(q1R))/4503599627370496)))/42535295865117307932921825928971026432 - (9007199067919185*cos(q3R)*((4774755754024928798560446539205*sin(q2R))/10141204801825835211973625643008 + cos(q2R)*((1211728953682539*cos(q1R))/2251799813685248 - (3148506117433717*sin(q1R))/4503599627370496) + (7514214926474921*sin(q2R)*((3148506117433717*cos(q1R))/4503599627370496 + (1211728953682539*sin(q1R))/2251799813685248))/36893488147419103232))/9007199254740992 + (67682029681889335677290557259385*sin(q3R)*((4774755754024928798560446539205*cos(q2R))/10141204801825835211973625643008 + (7514214926474921*cos(q2R)*((3148506117433717*cos(q1R))/4503599627370496 + (1211728953682539*sin(q1R))/2251799813685248))/36893488147419103232 - sin(q2R)*((1211728953682539*cos(q1R))/2251799813685248 - (3148506117433717*sin(q1R))/4503599627370496)))/332306998946228968225951765070086144 + (234819211581865*sin(q3R)*((4774755754024928798560446539205*sin(q2R))/10141204801825835211973625643008 + cos(q2R)*((1211728953682539*cos(q1R))/2251799813685248 - (3148506117433717*sin(q1R))/4503599627370496) + (7514214926474921*sin(q2R)*((3148506117433717*cos(q1R))/4503599627370496 + (1211728953682539*sin(q1R))/2251799813685248))/36893488147419103232))/1152921504606846976 + (2115063383689692319117831580025*cos(q3R)*((28359221366286827792295350160645*cos(q1R))/40564819207303340847894502572032 + (10914283902180054573281797610715*sin(q1R))/20282409603651670423947251286016 - 3983318308679801924058395430653/41538374868278621028243970633760768))/10384593717069655257060992658440192 + (81129635049124235038645691064225*sin(q3R)*((28359221366286827792295350160645*cos(q1R))/40564819207303340847894502572032 + (10914283902180054573281797610715*sin(q1R))/20282409603651670423947251286016 - 3983318308679801924058395430653/41538374868278621028243970633760768))/81129638414606681695789005144064))/119726214130147567059245861496117904970213993920593920 + (324259171862923063*sin(q6R)*((7514214926474921*sin(q5R)*(((4503599440548691*cos(q4R))/4503599627370496 - (7514214926474921*sin(q4R))/36893488147419103232)*((7514214926474921*cos(q3R)*((4774755754024928798560446539205*cos(q2R))/10141204801825835211973625643008 + (7514214926474921*cos(q2R)*((3148506117433717*cos(q1R))/4503599627370496 + (1211728953682539*sin(q1R))/2251799813685248))/36893488147419103232 - sin(q2R)*((1211728953682539*cos(q1R))/2251799813685248 - (3148506117433717*sin(q1R))/4503599627370496)))/36893488147419103232 + sin(q3R)*((4774755754024928798560446539205*sin(q2R))/10141204801825835211973625643008 + cos(q2R)*((1211728953682539*cos(q1R))/2251799813685248 - (3148506117433717*sin(q1R))/4503599627370496) + (7514214926474921*sin(q2R)*((3148506117433717*cos(q1R))/4503599627370496 + (1211728953682539*sin(q1R))/2251799813685248))/36893488147419103232) + (9007199067919185*cos(q3R)*((28359221366286827792295350160645*cos(q1R))/40564819207303340847894502572032 + (10914283902180054573281797610715*sin(q1R))/20282409603651670423947251286016 - 3983318308679801924058395430653/41538374868278621028243970633760768))/9007199254740992) - (7514214926474921*cos(q4R)*((7514214926474921*sin(q3R)*((4774755754024928798560446539205*cos(q2R))/10141204801825835211973625643008 + (7514214926474921*cos(q2R)*((3148506117433717*cos(q1R))/4503599627370496 + (1211728953682539*sin(q1R))/2251799813685248))/36893488147419103232 - sin(q2R)*((1211728953682539*cos(q1R))/2251799813685248 - (3148506117433717*sin(q1R))/4503599627370496)))/36893488147419103232 - cos(q3R)*((4774755754024928798560446539205*sin(q2R))/10141204801825835211973625643008 + cos(q2R)*((1211728953682539*cos(q1R))/2251799813685248 - (3148506117433717*sin(q1R))/4503599627370496) + (7514214926474921*sin(q2R)*((3148506117433717*cos(q1R))/4503599627370496 + (1211728953682539*sin(q1R))/2251799813685248))/36893488147419103232) + (9007199067919185*sin(q3R)*((28359221366286827792295350160645*cos(q1R))/40564819207303340847894502572032 + (10914283902180054573281797610715*sin(q1R))/20282409603651670423947251286016 - 3983318308679801924058395430653/41538374868278621028243970633760768))/9007199254740992))/36893488147419103232))/36893488147419103232 + cos(q5R)*((7514214926474921*sin(q4R)*((7514214926474921*sin(q3R)*((4774755754024928798560446539205*cos(q2R))/10141204801825835211973625643008 + (7514214926474921*cos(q2R)*((3148506117433717*cos(q1R))/4503599627370496 + (1211728953682539*sin(q1R))/2251799813685248))/36893488147419103232 - sin(q2R)*((1211728953682539*cos(q1R))/2251799813685248 - (3148506117433717*sin(q1R))/4503599627370496)))/36893488147419103232 - cos(q3R)*((4774755754024928798560446539205*sin(q2R))/10141204801825835211973625643008 + cos(q2R)*((1211728953682539*cos(q1R))/2251799813685248 - (3148506117433717*sin(q1R))/4503599627370496) + (7514214926474921*sin(q2R)*((3148506117433717*cos(q1R))/4503599627370496 + (1211728953682539*sin(q1R))/2251799813685248))/36893488147419103232) + (9007199067919185*sin(q3R)*((28359221366286827792295350160645*cos(q1R))/40564819207303340847894502572032 + (10914283902180054573281797610715*sin(q1R))/20282409603651670423947251286016 - 3983318308679801924058395430653/41538374868278621028243970633760768))/9007199254740992))/36893488147419103232 - ((7514214926474921*cos(q4R))/36893488147419103232 + (4503599440548691*sin(q4R))/4503599627370496)*((7514214926474921*cos(q3R)*((4774755754024928798560446539205*cos(q2R))/10141204801825835211973625643008 + (7514214926474921*cos(q2R)*((3148506117433717*cos(q1R))/4503599627370496 + (1211728953682539*sin(q1R))/2251799813685248))/36893488147419103232 - sin(q2R)*((1211728953682539*cos(q1R))/2251799813685248 - (3148506117433717*sin(q1R))/4503599627370496)))/36893488147419103232 + sin(q3R)*((4774755754024928798560446539205*sin(q2R))/10141204801825835211973625643008 + cos(q2R)*((1211728953682539*cos(q1R))/2251799813685248 - (3148506117433717*sin(q1R))/4503599627370496) + (7514214926474921*sin(q2R)*((3148506117433717*cos(q1R))/4503599627370496 + (1211728953682539*sin(q1R))/2251799813685248))/36893488147419103232) + (9007199067919185*cos(q3R)*((28359221366286827792295350160645*cos(q1R))/40564819207303340847894502572032 + (10914283902180054573281797610715*sin(q1R))/20282409603651670423947251286016 - 3983318308679801924058395430653/41538374868278621028243970633760768))/9007199254740992)) - (9007199067919185*sin(q5R)*((1764482024691522628700660907665*cos(q3R)*((4774755754024928798560446539205*cos(q2R))/10141204801825835211973625643008 + (7514214926474921*cos(q2R)*((3148506117433717*cos(q1R))/4503599627370496 + (1211728953682539*sin(q1R))/2251799813685248))/36893488147419103232 - sin(q2R)*((1211728953682539*cos(q1R))/2251799813685248 - (3148506117433717*sin(q1R))/4503599627370496)))/42535295865117307932921825928971026432 - (9007199067919185*cos(q3R)*((4774755754024928798560446539205*sin(q2R))/10141204801825835211973625643008 + cos(q2R)*((1211728953682539*cos(q1R))/2251799813685248 - (3148506117433717*sin(q1R))/4503599627370496) + (7514214926474921*sin(q2R)*((3148506117433717*cos(q1R))/4503599627370496 + (1211728953682539*sin(q1R))/2251799813685248))/36893488147419103232))/9007199254740992 + (67682029681889335677290557259385*sin(q3R)*((4774755754024928798560446539205*cos(q2R))/10141204801825835211973625643008 + (7514214926474921*cos(q2R)*((3148506117433717*cos(q1R))/4503599627370496 + (1211728953682539*sin(q1R))/2251799813685248))/36893488147419103232 - sin(q2R)*((1211728953682539*cos(q1R))/2251799813685248 - (3148506117433717*sin(q1R))/4503599627370496)))/332306998946228968225951765070086144 + (234819211581865*sin(q3R)*((4774755754024928798560446539205*sin(q2R))/10141204801825835211973625643008 + cos(q2R)*((1211728953682539*cos(q1R))/2251799813685248 - (3148506117433717*sin(q1R))/4503599627370496) + (7514214926474921*sin(q2R)*((3148506117433717*cos(q1R))/4503599627370496 + (1211728953682539*sin(q1R))/2251799813685248))/36893488147419103232))/1152921504606846976 + (2115063383689692319117831580025*cos(q3R)*((28359221366286827792295350160645*cos(q1R))/40564819207303340847894502572032 + (10914283902180054573281797610715*sin(q1R))/20282409603651670423947251286016 - 3983318308679801924058395430653/41538374868278621028243970633760768))/10384593717069655257060992658440192 + (81129635049124235038645691064225*sin(q3R)*((28359221366286827792295350160645*cos(q1R))/40564819207303340847894502572032 + (10914283902180054573281797610715*sin(q1R))/20282409603651670423947251286016 - 3983318308679801924058395430653/41538374868278621028243970633760768))/81129638414606681695789005144064))/9007199254740992))/9007199254740992000 - (610321541873521657855151997354401418608858870661075444886782706002880706727*cos(q4R)*((7514214926474921*sin(q3R)*((4774755754024928798560446539205*cos(q2R))/10141204801825835211973625643008 + (7514214926474921*cos(q2R)*((3148506117433717*cos(q1R))/4503599627370496 + (1211728953682539*sin(q1R))/2251799813685248))/36893488147419103232 - sin(q2R)*((1211728953682539*cos(q1R))/2251799813685248 - (3148506117433717*sin(q1R))/4503599627370496)))/36893488147419103232 - cos(q3R)*((4774755754024928798560446539205*sin(q2R))/10141204801825835211973625643008 + cos(q2R)*((1211728953682539*cos(q1R))/2251799813685248 - (3148506117433717*sin(q1R))/4503599627370496) + (7514214926474921*sin(q2R)*((3148506117433717*cos(q1R))/4503599627370496 + (1211728953682539*sin(q1R))/2251799813685248))/36893488147419103232) + (9007199067919185*sin(q3R)*((28359221366286827792295350160645*cos(q1R))/40564819207303340847894502572032 + (10914283902180054573281797610715*sin(q1R))/20282409603651670423947251286016 - 3983318308679801924058395430653/41538374868278621028243970633760768))/9007199254740992))/11307821214581659709333104004754678501295896940003961331978279688272766566400000 + (83301539375654672537075965313343183841442266989297270401707771044036658496661398777306991*sin(q3R)*((28359221366286827792295350160645*cos(q1R))/40564819207303340847894502572032 + (10914283902180054573281797610715*sin(q1R))/20282409603651670423947251286016 - 3983318308679801924058395430653/41538374868278621028243970633760768))/4074071952668972172536891376818756322102936787331872501272280898708762599526673412366794752000 - (48638874966763599*sin(q5R)*((1764482024691522628700660907665*cos(q3R)*((4774755754024928798560446539205*cos(q2R))/10141204801825835211973625643008 + (7514214926474921*cos(q2R)*((3148506117433717*cos(q1R))/4503599627370496 + (1211728953682539*sin(q1R))/2251799813685248))/36893488147419103232 - sin(q2R)*((1211728953682539*cos(q1R))/2251799813685248 - (3148506117433717*sin(q1R))/4503599627370496)))/42535295865117307932921825928971026432 - (9007199067919185*cos(q3R)*((4774755754024928798560446539205*sin(q2R))/10141204801825835211973625643008 + cos(q2R)*((1211728953682539*cos(q1R))/2251799813685248 - (3148506117433717*sin(q1R))/4503599627370496) + (7514214926474921*sin(q2R)*((3148506117433717*cos(q1R))/4503599627370496 + (1211728953682539*sin(q1R))/2251799813685248))/36893488147419103232))/9007199254740992 + (67682029681889335677290557259385*sin(q3R)*((4774755754024928798560446539205*cos(q2R))/10141204801825835211973625643008 + (7514214926474921*cos(q2R)*((3148506117433717*cos(q1R))/4503599627370496 + (1211728953682539*sin(q1R))/2251799813685248))/36893488147419103232 - sin(q2R)*((1211728953682539*cos(q1R))/2251799813685248 - (3148506117433717*sin(q1R))/4503599627370496)))/332306998946228968225951765070086144 + (234819211581865*sin(q3R)*((4774755754024928798560446539205*sin(q2R))/10141204801825835211973625643008 + cos(q2R)*((1211728953682539*cos(q1R))/2251799813685248 - (3148506117433717*sin(q1R))/4503599627370496) + (7514214926474921*sin(q2R)*((3148506117433717*cos(q1R))/4503599627370496 + (1211728953682539*sin(q1R))/2251799813685248))/36893488147419103232))/1152921504606846976 + (2115063383689692319117831580025*cos(q3R)*((28359221366286827792295350160645*cos(q1R))/40564819207303340847894502572032 + (10914283902180054573281797610715*sin(q1R))/20282409603651670423947251286016 - 3983318308679801924058395430653/41538374868278621028243970633760768))/10384593717069655257060992658440192 + (81129635049124235038645691064225*sin(q3R)*((28359221366286827792295350160645*cos(q1R))/40564819207303340847894502572032 + (10914283902180054573281797610715*sin(q1R))/20282409603651670423947251286016 - 3983318308679801924058395430653/41538374868278621028243970633760768))/81129638414606681695789005144064))/1801439850948198400, (202883803014822867*sin(q6R)*(sin(q5R)*(((4503599440548691*cos(q4R))/4503599627370496 - (7514214926474921*sin(q4R))/36893488147419103232)*((7514214926474921*sin(q3R)*((4774755754024928798560446539205*cos(q2R))/10141204801825835211973625643008 + (7514214926474921*cos(q2R)*((3148506117433717*cos(q1R))/4503599627370496 + (1211728953682539*sin(q1R))/2251799813685248))/36893488147419103232 - sin(q2R)*((1211728953682539*cos(q1R))/2251799813685248 - (3148506117433717*sin(q1R))/4503599627370496)))/36893488147419103232 - cos(q3R)*((4774755754024928798560446539205*sin(q2R))/10141204801825835211973625643008 + cos(q2R)*((1211728953682539*cos(q1R))/2251799813685248 - (3148506117433717*sin(q1R))/4503599627370496) + (7514214926474921*sin(q2R)*((3148506117433717*cos(q1R))/4503599627370496 + (1211728953682539*sin(q1R))/2251799813685248))/36893488147419103232) + (9007199067919185*sin(q3R)*((28359221366286827792295350160645*cos(q1R))/40564819207303340847894502572032 + (10914283902180054573281797610715*sin(q1R))/20282409603651670423947251286016 - 3983318308679801924058395430653/41538374868278621028243970633760768))/9007199254740992) + ((234819211581865*cos(q4R))/1152921504606846976 + (9007199067919185*sin(q4R))/9007199254740992)*((213097284493758984364555654519459856780913684045*cos(q1R))/1496577676626844588240573268701473812127674924007424 - (43007175577195104036898489188735438973874147925*cos(q2R))/91343852333181432387730302044767688728495783936 + (82012275009546312639155898108543355135168378515*sin(q1R))/748288838313422294120286634350736906063837462003712 - (67682029681889335677290557259385*cos(q2R)*((3148506117433717*cos(q1R))/4503599627370496 + (1211728953682539*sin(q1R))/2251799813685248))/332306998946228968225951765070086144 + (9007199067919185*sin(q2R)*((1211728953682539*cos(q1R))/2251799813685248 - (3148506117433717*sin(q1R))/4503599627370496))/9007199254740992 - 29931509891982604486959633650198707742999153413/1532495540865888858358347027150309183618739122183602176) + (7514214926474921*cos(q4R)*((7514214926474921*cos(q3R)*((4774755754024928798560446539205*cos(q2R))/10141204801825835211973625643008 + (7514214926474921*cos(q2R)*((3148506117433717*cos(q1R))/4503599627370496 + (1211728953682539*sin(q1R))/2251799813685248))/36893488147419103232 - sin(q2R)*((1211728953682539*cos(q1R))/2251799813685248 - (3148506117433717*sin(q1R))/4503599627370496)))/36893488147419103232 + sin(q3R)*((4774755754024928798560446539205*sin(q2R))/10141204801825835211973625643008 + cos(q2R)*((1211728953682539*cos(q1R))/2251799813685248 - (3148506117433717*sin(q1R))/4503599627370496) + (7514214926474921*sin(q2R)*((3148506117433717*cos(q1R))/4503599627370496 + (1211728953682539*sin(q1R))/2251799813685248))/36893488147419103232) + (9007199067919185*cos(q3R)*((28359221366286827792295350160645*cos(q1R))/40564819207303340847894502572032 + (10914283902180054573281797610715*sin(q1R))/20282409603651670423947251286016 - 3983318308679801924058395430653/41538374868278621028243970633760768))/9007199254740992))/36893488147419103232) - (7514214926474921*cos(q5R)*(((7514214926474921*cos(q4R))/36893488147419103232 + (4503599440548691*sin(q4R))/4503599627370496)*((7514214926474921*sin(q3R)*((4774755754024928798560446539205*cos(q2R))/10141204801825835211973625643008 + (7514214926474921*cos(q2R)*((3148506117433717*cos(q1R))/4503599627370496 + (1211728953682539*sin(q1R))/2251799813685248))/36893488147419103232 - sin(q2R)*((1211728953682539*cos(q1R))/2251799813685248 - (3148506117433717*sin(q1R))/4503599627370496)))/36893488147419103232 - cos(q3R)*((4774755754024928798560446539205*sin(q2R))/10141204801825835211973625643008 + cos(q2R)*((1211728953682539*cos(q1R))/2251799813685248 - (3148506117433717*sin(q1R))/4503599627370496) + (7514214926474921*sin(q2R)*((3148506117433717*cos(q1R))/4503599627370496 + (1211728953682539*sin(q1R))/2251799813685248))/36893488147419103232) + (9007199067919185*sin(q3R)*((28359221366286827792295350160645*cos(q1R))/40564819207303340847894502572032 + (10914283902180054573281797610715*sin(q1R))/20282409603651670423947251286016 - 3983318308679801924058395430653/41538374868278621028243970633760768))/9007199254740992) - ((9007199067919185*cos(q4R))/9007199254740992 - (234819211581865*sin(q4R))/1152921504606846976)*((213097284493758984364555654519459856780913684045*cos(q1R))/1496577676626844588240573268701473812127674924007424 - (43007175577195104036898489188735438973874147925*cos(q2R))/91343852333181432387730302044767688728495783936 + (82012275009546312639155898108543355135168378515*sin(q1R))/748288838313422294120286634350736906063837462003712 - (67682029681889335677290557259385*cos(q2R)*((3148506117433717*cos(q1R))/4503599627370496 + (1211728953682539*sin(q1R))/2251799813685248))/332306998946228968225951765070086144 + (9007199067919185*sin(q2R)*((1211728953682539*cos(q1R))/2251799813685248 - (3148506117433717*sin(q1R))/4503599627370496))/9007199254740992 - 29931509891982604486959633650198707742999153413/1532495540865888858358347027150309183618739122183602176) + (7514214926474921*sin(q4R)*((7514214926474921*cos(q3R)*((4774755754024928798560446539205*cos(q2R))/10141204801825835211973625643008 + (7514214926474921*cos(q2R)*((3148506117433717*cos(q1R))/4503599627370496 + (1211728953682539*sin(q1R))/2251799813685248))/36893488147419103232 - sin(q2R)*((1211728953682539*cos(q1R))/2251799813685248 - (3148506117433717*sin(q1R))/4503599627370496)))/36893488147419103232 + sin(q3R)*((4774755754024928798560446539205*sin(q2R))/10141204801825835211973625643008 + cos(q2R)*((1211728953682539*cos(q1R))/2251799813685248 - (3148506117433717*sin(q1R))/4503599627370496) + (7514214926474921*sin(q2R)*((3148506117433717*cos(q1R))/4503599627370496 + (1211728953682539*sin(q1R))/2251799813685248))/36893488147419103232) + (9007199067919185*cos(q3R)*((28359221366286827792295350160645*cos(q1R))/40564819207303340847894502572032 + (10914283902180054573281797610715*sin(q1R))/20282409603651670423947251286016 - 3983318308679801924058395430653/41538374868278621028243970633760768))/9007199254740992))/36893488147419103232))/36893488147419103232))/36893488147419103232000 - (202883803014822867*sin(q5R)*(((7514214926474921*cos(q4R))/36893488147419103232 + (4503599440548691*sin(q4R))/4503599627370496)*((7514214926474921*sin(q3R)*((4774755754024928798560446539205*cos(q2R))/10141204801825835211973625643008 + (7514214926474921*cos(q2R)*((3148506117433717*cos(q1R))/4503599627370496 + (1211728953682539*sin(q1R))/2251799813685248))/36893488147419103232 - sin(q2R)*((1211728953682539*cos(q1R))/2251799813685248 - (3148506117433717*sin(q1R))/4503599627370496)))/36893488147419103232 - cos(q3R)*((4774755754024928798560446539205*sin(q2R))/10141204801825835211973625643008 + cos(q2R)*((1211728953682539*cos(q1R))/2251799813685248 - (3148506117433717*sin(q1R))/4503599627370496) + (7514214926474921*sin(q2R)*((3148506117433717*cos(q1R))/4503599627370496 + (1211728953682539*sin(q1R))/2251799813685248))/36893488147419103232) + (9007199067919185*sin(q3R)*((28359221366286827792295350160645*cos(q1R))/40564819207303340847894502572032 + (10914283902180054573281797610715*sin(q1R))/20282409603651670423947251286016 - 3983318308679801924058395430653/41538374868278621028243970633760768))/9007199254740992) - ((9007199067919185*cos(q4R))/9007199254740992 - (234819211581865*sin(q4R))/1152921504606846976)*((213097284493758984364555654519459856780913684045*cos(q1R))/1496577676626844588240573268701473812127674924007424 - (43007175577195104036898489188735438973874147925*cos(q2R))/91343852333181432387730302044767688728495783936 + (82012275009546312639155898108543355135168378515*sin(q1R))/748288838313422294120286634350736906063837462003712 - (67682029681889335677290557259385*cos(q2R)*((3148506117433717*cos(q1R))/4503599627370496 + (1211728953682539*sin(q1R))/2251799813685248))/332306998946228968225951765070086144 + (9007199067919185*sin(q2R)*((1211728953682539*cos(q1R))/2251799813685248 - (3148506117433717*sin(q1R))/4503599627370496))/9007199254740992 - 29931509891982604486959633650198707742999153413/1532495540865888858358347027150309183618739122183602176) + (7514214926474921*sin(q4R)*((7514214926474921*cos(q3R)*((4774755754024928798560446539205*cos(q2R))/10141204801825835211973625643008 + (7514214926474921*cos(q2R)*((3148506117433717*cos(q1R))/4503599627370496 + (1211728953682539*sin(q1R))/2251799813685248))/36893488147419103232 - sin(q2R)*((1211728953682539*cos(q1R))/2251799813685248 - (3148506117433717*sin(q1R))/4503599627370496)))/36893488147419103232 + sin(q3R)*((4774755754024928798560446539205*sin(q2R))/10141204801825835211973625643008 + cos(q2R)*((1211728953682539*cos(q1R))/2251799813685248 - (3148506117433717*sin(q1R))/4503599627370496) + (7514214926474921*sin(q2R)*((3148506117433717*cos(q1R))/4503599627370496 + (1211728953682539*sin(q1R))/2251799813685248))/36893488147419103232) + (9007199067919185*cos(q3R)*((28359221366286827792295350160645*cos(q1R))/40564819207303340847894502572032 + (10914283902180054573281797610715*sin(q1R))/20282409603651670423947251286016 - 3983318308679801924058395430653/41538374868278621028243970633760768))/9007199254740992))/36893488147419103232))/36893488147419103232000 - (324259171862923063*sin(q6R)*((7514214926474921*sin(q5R)*(((7514214926474921*cos(q4R))/36893488147419103232 + 